simulink model "SSN_39busRT_Ctrl_4WT_19B"  (R2021a)
settings: Solver=ode3  StartTime=0.0  StopTime=10  FixedStep=Ts  MaxStep=1/60  RelTol=1e-2  AbsTol=1e-1
PreLoadFcn:
  | Ts=2.50e-6; ssn_ieee39_params; load('Pwf.mat');
InitFcn:
  | Ts=2.50e-6; ssn_ieee39_params; load('Pwf.mat');
values from neighbouring files (symbols this model uses):
  f = 50    [ssn_ieee39_params_ctrl.m]
  fNom = f    (= 60)    [ssn_ieee39_params_ctrl.m]
  ILR = 5.02    [ssn_ieee39_params_ctrl.m]
  IQMIN = 0.1    [ssn_ieee39_params_ctrl.m]
  ISCLIM = 1    [ssn_ieee39_params_ctrl.m]
  ITFpu = 1.10    (= 1.1)    [ssn_ieee39_params_ctrl.m]
  K = 1    [ssn_ieee39_params_ctrl.m]
  K1 = 1    [ssn_ieee39_params_ctrl.m]
  K2 = 2    [ssn_ieee39_params_ctrl.m]
  KCL = 1.04    [ssn_ieee39_params_ctrl.m]
  KFB = 0    [ssn_ieee39_params_ctrl.m]
  KFF = 1    [ssn_ieee39_params_ctrl.m]
  KFIX = 1    [ssn_ieee39_params_ctrl.m]
  KG = 1    [ssn_ieee39_params_ctrl.m]
  KIA = 59.91    [ssn_ieee39_params_ctrl.m]
  KIOEX = 0.0303    [ssn_ieee39_params_ctrl.m]
  KIUEX = 0.0303    [ssn_ieee39_params_ctrl.m]
  KIUOEX = 1    [ssn_ieee39_params_ctrl.m]
  KIUUEX = 1    [ssn_ieee39_params_ctrl.m]
  KLR = 22.47    [ssn_ieee39_params_ctrl.m]
  KM = 1    [ssn_ieee39_params_ctrl.m]
  KOEL = 0.24    [ssn_ieee39_params_ctrl.m]
  Kp = 1    [ssn_ieee39_params_ctrl.m]
  KPA = 30    [ssn_ieee39_params_ctrl.m]
  KPOEL = 1    [ssn_ieee39_params_ctrl.m]
  KPOEX = 0    [ssn_ieee39_params_ctrl.m]
  KPUEX = 0    [ssn_ieee39_params_ctrl.m]
  KSCALE = 0.319    [ssn_ieee39_params_ctrl.m]
  KUF = 0    [ssn_ieee39_params_ctrl.m]
  KUI = 0.001    [ssn_ieee39_params_ctrl.m]
  KUL = 0.24    [ssn_ieee39_params_ctrl.m]
  s = 10    [ssn_ieee39_params_ctrl.m]
  TA = 0.01    [ssn_ieee39_params_ctrl.m]
  Tadj = 0    [ssn_ieee39_params_ctrl.m]
  taps = [1 1 1.07 1.07 1.009 1.025 1 1.025 1.025 1.025]*1    [ssn_ieee39_params_ctrl.m]
  TF = 0.02    [ssn_ieee39_params_ctrl.m]
  TG = 0.024    [ssn_ieee39_params_ctrl.m]
  TINV = 0    [ssn_ieee39_params_ctrl.m]
  TIT = 0.1    [ssn_ieee39_params_ctrl.m]
  TL_10_11_len = 14    [ssn_ieee39_params_ctrl.m]
  TL_10_13_len = 14    [ssn_ieee39_params_ctrl.m]
  TL_13_14_len = 32    [ssn_ieee39_params_ctrl.m]
  TL_14_15_len = 70    [ssn_ieee39_params_ctrl.m]
  TL_15_16_len = 31.5    [ssn_ieee39_params_ctrl.m]
  TL_16_17_len = 26    [ssn_ieee39_params_ctrl.m]
  TL_16_19_len = 61    [ssn_ieee39_params_ctrl.m]
  TL_16_21_len = 46    [ssn_ieee39_params_ctrl.m]
  TL_16_24_len = 15    [ssn_ieee39_params_ctrl.m]
  TL_17_18_len = 26    [ssn_ieee39_params_ctrl.m]
  TL_17_27_len = 59    [ssn_ieee39_params_ctrl.m]
  TL_1_2_len = 134    [ssn_ieee39_params_ctrl.m]
  TL_1_39_len = 105    [ssn_ieee39_params_ctrl.m]
  TL_21_22_len = 47    [ssn_ieee39_params_ctrl.m]
  TL_22_23_len = 33    [ssn_ieee39_params_ctrl.m]
  TL_24_23_len = 88    [ssn_ieee39_params_ctrl.m]
  TL_25_26_len = 101    [ssn_ieee39_params_ctrl.m]
  TL_26_27_len = 46.5    [ssn_ieee39_params_ctrl.m]
  TL_26_28_len = 151    [ssn_ieee39_params_ctrl.m]
  TL_26_29_len = 200    [ssn_ieee39_params_ctrl.m]
  TL_28_29_len = 48    [ssn_ieee39_params_ctrl.m]
  TL_2_25_len = 28    [ssn_ieee39_params_ctrl.m]
  TL_2_2_len = 49    [ssn_ieee39_params_ctrl.m]
  TL_3_18_len = 42    [ssn_ieee39_params_ctrl.m]
  TL_3_4_len = 53    [ssn_ieee39_params_ctrl.m]
  TL_4_14_len = 33    [ssn_ieee39_params_ctrl.m]
  TL_4_5_len = 32.5    [ssn_ieee39_params_ctrl.m]
  TL_5_6_len = 14    [ssn_ieee39_params_ctrl.m]
  TL_5_8_len = 32    [ssn_ieee39_params_ctrl.m]
  TL_6_11_len = 26.5    [ssn_ieee39_params_ctrl.m]
  TL_6_7_len = 25.5    [ssn_ieee39_params_ctrl.m]
  TL_7_8_len = 15    [ssn_ieee39_params_ctrl.m]
  TL_8_9_len = 93    [ssn_ieee39_params_ctrl.m]
  TL_9_39_len = 136    [ssn_ieee39_params_ctrl.m]
  TOEL = 5.00    (= 5)    [ssn_ieee39_params_ctrl.m]
  TQREF = 0    [ssn_ieee39_params_ctrl.m]
  TQSCL = 0.012    [ssn_ieee39_params_ctrl.m]
  Ts_PMU = 1/1000    (= 0.001)    [ssn_ieee39_params_ctrl.m]
  TU1 = 0    [ssn_ieee39_params_ctrl.m]
  TU2 = 0    [ssn_ieee39_params_ctrl.m]
  TU3 = 0    [ssn_ieee39_params_ctrl.m]
  TU4 = 0    [ssn_ieee39_params_ctrl.m]
  TUL = 0    [ssn_ieee39_params_ctrl.m]
  TUP = 0.050    (= 0.05)    [ssn_ieee39_params_ctrl.m]
  TUQ = .005    (= 0.005)    [ssn_ieee39_params_ctrl.m]
  TUV = 0.2    [ssn_ieee39_params_ctrl.m]
  VAAMAX = VAMAX    (= 7.05)    [ssn_ieee39_params_ctrl.m]
  VAMAX = 7.05    [ssn_ieee39_params_ctrl.m]
  VAMIN = -6.11    [ssn_ieee39_params_ctrl.m]
  VBMAX = 999    [ssn_ieee39_params_ctrl.m]
  VF = 0    [ssn_ieee39_params_ctrl.m]
  VFB = 0    [ssn_ieee39_params_ctrl.m]
  VMMAX = 7.05    [ssn_ieee39_params_ctrl.m]
  VMMIN = -6.11    [ssn_ieee39_params_ctrl.m]
  VOELmax1 = 0.2353    [ssn_ieee39_params_ctrl.m]
  VOELmax2 = 0.0    (= 0)    [ssn_ieee39_params_ctrl.m]
  VOELmin1 = -0.24    [ssn_ieee39_params_ctrl.m]
  VOELmin2 = -1.0    (= -1)    [ssn_ieee39_params_ctrl.m]
  VRMAX = 7.05    [ssn_ieee39_params_ctrl.m]
  VRMIN = -6.11    [ssn_ieee39_params_ctrl.m]
  VSCLmax = 0.20    (= 0.2)    [ssn_ieee39_params_ctrl.m]
  VSCLmin = -0.10    (= -0.1)    [ssn_ieee39_params_ctrl.m]
  VUELmax1 = 1    [ssn_ieee39_params_ctrl.m]
  VUELmax2 = 1    [ssn_ieee39_params_ctrl.m]
  VUELmin1 = -1    [ssn_ieee39_params_ctrl.m]
  VUELmin2 = -1    [ssn_ieee39_params_ctrl.m]
  VUImax = 1    [ssn_ieee39_params_ctrl.m]
  VUImin = -1    [ssn_ieee39_params_ctrl.m]
undefined symbols (not defined in the file or in its folder): another_event_name, D1, Delta, DiscIntNeverNeededParam, find_system, MOV_segment9, my_event_name, powergui, Pw1, Pw2, Pw3, Pw4, vNomHV
libraries: powerlib_extras x162, spsThreePhaseVIMeasurementLib x55, spsCurrentMeasurementLib x52, simulink_extras x44, slpidlib x40, op_dpl_lib x36, spsST2AModel x20, spsThreePhaseParallelRLCLoadLib x20, spsThreePhaseTransformerTwoWindingsLib x17, spsControlledVoltageSourceLib x16, spsVoltageMeasurementLib x12, spsSynchronousMachinepuStandardLib x10
(part 2 of 19)

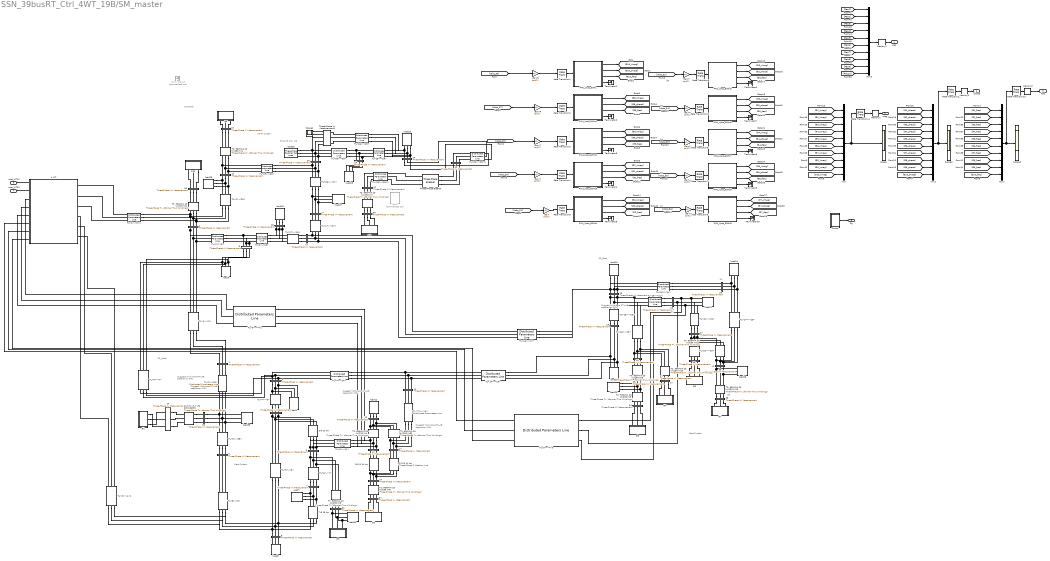
== system SSN_39busRT_Ctrl_4WT_19B/SM_master ==
  note: SS_East
  note: SM_North
  note: SS_West
  note: West System
  note: Suggest multi-core
      | RT-LAB separation DPL
  note: Suggest Multi-core
      | RT-LAB separation DPL
  note: Suggest Multi-core
      | RT-LAB separation DPL
  note: Suggest Multi-core
      | RT-LAB separation DPL
  note: P&Q 29 ==> 26
  note: North System
  note: 33
  note: 21
  note: 24
  note: 36
  note: 23
  note: Suggest Multi-core
      | RT-LAB separation DPL
  note: East System
  note: G3
  note: G7
  note: G6
  note: G4
  note: G5
  1 : spsThreePhaseVIMeasurementLib/Three-Phase V-I Measurement  VoltageMeasurement=phase-to-phase  SetLabelV=on  LabelV=Vabc_1  Vpu=off  VpuLL=on  CurrentMeasurement=no  SetLabelI=on  LabelI=Iabc_B2  Ipu=off  Pbase=100e6  Vbase=Bus(1,2)*1e3  OutputType=Complex  PhasorSimulation=off  PSBequivalent=0
  10 : spsThreePhaseVIMeasurementLib/Three-Phase V-I Measurement  VoltageMeasurement=phase-to-phase  SetLabelV=on  LabelV=Vabc_10  Vpu=off  VpuLL=on  CurrentMeasurement=no  SetLabelI=on  LabelI=Iabc_B2  Ipu=off  Pbase=100e6  Vbase=Bus(10,2)*1e3  OutputType=Complex  PhasorSimulation=off  PSBequivalent=0
  10-11 14 km : spsThreePhasePISectionLineLib/Three-Phase PI Section Line  LConnTagsString=a|b|c  RConnTagsString=A|B|C  Length=TL_10_11_len  Frequency=60  Resistances=[0.476 1.904]/TL_10_11_len  Inductances="[0.014  0.04]/TL_10_11_len"  Capacitances=[0.162e-6 0.074e-6]/TL_10_11_len
  10-13 14 km : spsThreePhasePISectionLineLib/Three-Phase PI Section Line  LConnTagsString=a|b|c  RConnTagsString=A|B|C  Length=TL_10_13_len  Frequency=60  Resistances=[0.476 1.904]/TL_10_13_len  Inductances="[0.014  0.04]/TL_10_13_len"  Capacitances=[0.162e-6 0.074e-6]/TL_10_13_len
  11 : spsThreePhaseVIMeasurementLib/Three-Phase V-I Measurement  VoltageMeasurement=phase-to-phase  SetLabelV=on  LabelV=Vabc_11  Vpu=off  VpuLL=on  CurrentMeasurement=no  SetLabelI=on  LabelI=Iabc_B2  Ipu=off  Pbase=100e6  Vbase=Bus(11,2)*1e3  OutputType=Complex  PhasorSimulation=off  PSBequivalent=0
  12 : spsThreePhaseVIMeasurementLib/Three-Phase V-I Measurement  VoltageMeasurement=phase-to-phase  SetLabelV=on  LabelV=Vabc_12  Vpu=off  VpuLL=on  CurrentMeasurement=no  SetLabelI=on  LabelI=Iabc_B2  Ipu=off  Pbase=100e6  Vbase=Bus(12,2)*1e3  OutputType=Complex  PhasorSimulation=off  PSBequivalent=0
  13 : spsThreePhaseVIMeasurementLib/Three-Phase V-I Measurement  VoltageMeasurement=phase-to-phase  SetLabelV=on  LabelV=Vabc_13  Vpu=off  VpuLL=on  CurrentMeasurement=no  SetLabelI=on  LabelI=Iabc_B2  Ipu=off  Pbase=100e6  Vbase=Bus(13,2)*1e3  OutputType=Complex  PhasorSimulation=off  PSBequivalent=0
  14 : spsThreePhaseVIMeasurementLib/Three-Phase V-I Measurement  VoltageMeasurement=phase-to-phase  SetLabelV=on  LabelV=Vabc_14  Vpu=off  VpuLL=on  CurrentMeasurement=no  SetLabelI=on  LabelI=Iabc_B2  Ipu=off  Pbase=100e6  Vbase=Bus(14,2)*1e3  OutputType=Complex  PhasorSimulation=off  PSBequivalent=0
  15 : spsThreePhaseVIMeasurementLib/Three-Phase V-I Measurement  VoltageMeasurement=phase-to-phase  SetLabelV=on  LabelV=Vabc_15  Vpu=off  VpuLL=on  CurrentMeasurement=no  SetLabelI=on  LabelI=Iabc_B2  Ipu=off  Pbase=100e6  Vbase=Bus(15,2)*1e3  OutputType=Complex  PhasorSimulation=off  PSBequivalent=0
  16 : spsThreePhaseVIMeasurementLib/Three-Phase V-I Measurement  VoltageMeasurement=phase-to-phase  SetLabelV=on  LabelV=Vabc_16  Vpu=off  VpuLL=on  CurrentMeasurement=no  SetLabelI=on  LabelI=Iabc_B2  Ipu=off  Pbase=100e6  Vbase=Bus(16,2)*1e3  OutputType=Complex  PhasorSimulation=off  PSBequivalent=0
  17 : spsThreePhaseVIMeasurementLib/Three-Phase V-I Measurement  VoltageMeasurement=phase-to-phase  SetLabelV=on  LabelV=Vabc_17  Vpu=off  VpuLL=on  CurrentMeasurement=no  SetLabelI=on  LabelI=Iabc_B2  Ipu=off  Pbase=100e6  Vbase=Bus(17,2)*1e3  OutputType=Complex  PhasorSimulation=off  PSBequivalent=0
  18 : spsThreePhaseVIMeasurementLib/Three-Phase V-I Measurement  VoltageMeasurement=phase-to-phase  SetLabelV=on  LabelV=Vabc_18  Vpu=off  VpuLL=on  CurrentMeasurement=no  SetLabelI=on  LabelI=Iabc_B2  Ipu=off  Pbase=100e6  Vbase=Bus(18,2)*1e3  OutputType=Complex  PhasorSimulation=off  PSBequivalent=0
  19 : spsThreePhaseVIMeasurementLib/Three-Phase V-I Measurement  VoltageMeasurement=phase-to-phase  SetLabelV=on  LabelV=Vabc_19  Vpu=off  VpuLL=on  CurrentMeasurement=no  SetLabelI=on  LabelI=Iabc_B2  Ipu=off  Pbase=100e6  Vbase=Bus(19,2)*1e3  OutputType=Complex  PhasorSimulation=off  PSBequivalent=0
  2 : spsThreePhaseVIMeasurementLib/Three-Phase V-I Measurement  VoltageMeasurement=phase-to-phase  SetLabelV=on  LabelV=Vabc_2  Vpu=off  VpuLL=on  CurrentMeasurement=no  SetLabelI=on  LabelI=Iabc_B2  Ipu=off  Pbase=100e6  Vbase=Bus(2,2)*1e3  OutputType=Complex  PhasorSimulation=off  PSBequivalent=0
  20 : spsThreePhaseVIMeasurementLib/Three-Phase V-I Measurement  VoltageMeasurement=phase-to-phase  SetLabelV=on  LabelV=Vabc_20  Vpu=off  VpuLL=on  CurrentMeasurement=no  SetLabelI=on  LabelI=Iabc_B2  Ipu=off  Pbase=100e6  Vbase=Bus(20,2)*1e3  OutputType=Complex  PhasorSimulation=off  PSBequivalent=0
  21 : spsThreePhaseVIMeasurementLib/Three-Phase V-I Measurement  VoltageMeasurement=phase-to-phase  SetLabelV=on  LabelV=Vabc_33  Vpu=off  VpuLL=on  CurrentMeasurement=yes  SetLabelI=on  LabelI=Iabc_33  Ipu=on  Pbase=1000e6  Vbase=Bus(33,2)*1e3  OutputType=Complex  PhasorSimulation=off  PSBequivalent=0
  22 : spsThreePhaseVIMeasurementLib/Three-Phase V-I Measurement  VoltageMeasurement=phase-to-phase  SetLabelV=on  LabelV=Vabc_22  Vpu=off  VpuLL=on  CurrentMeasurement=no  SetLabelI=on  LabelI=Iabc_B2  Ipu=off  Pbase=100e6  Vbase=Bus(22,2)*1e3  OutputType=Complex  PhasorSimulation=off  PSBequivalent=0
  23 : spsThreePhaseVIMeasurementLib/Three-Phase V-I Measurement  VoltageMeasurement=phase-to-phase  SetLabelV=on  LabelV=Vabc_21  Vpu=off  VpuLL=on  CurrentMeasurement=no  SetLabelI=on  LabelI=Iabc_B2  Ipu=off  Pbase=100e6  Vbase=Bus(21,2)*1e3  OutputType=Complex  PhasorSimulation=off  PSBequivalent=0
  24 : spsThreePhaseVIMeasurementLib/Three-Phase V-I Measurement  VoltageMeasurement=phase-to-phase  SetLabelV=on  LabelV=Vabc_391  Vpu=off  VpuLL=on  CurrentMeasurement=yes  SetLabelI=on  LabelI=Iabc_391  Ipu=on  Pbase=1000e6  Vbase=Bus(30,2)*1e3  OutputType=Complex  PhasorSimulation=off  PSBequivalent=0
  25 : spsThreePhaseVIMeasurementLib/Three-Phase V-I Measurement  VoltageMeasurement=phase-to-phase  SetLabelV=on  LabelV=Vabc_25  Vpu=off  VpuLL=on  CurrentMeasurement=no  SetLabelI=on  LabelI=Iabc_B2  Ipu=off  Pbase=100e6  Vbase=Bus(25,2)*1e3  OutputType=Complex  PhasorSimulation=off  PSBequivalent=0
  26 : spsThreePhaseVIMeasurementLib/Three-Phase V-I Measurement  VoltageMeasurement=phase-to-phase  SetLabelV=on  LabelV=Vabc_26  Vpu=off  VpuLL=on  CurrentMeasurement=no  SetLabelI=on  LabelI=Iabc_B2  Ipu=off  Pbase=100e6  Vbase=Bus(26,2)*1e3  OutputType=Complex  PhasorSimulation=off  PSBequivalent=0
  27 : spsThreePhaseVIMeasurementLib/Three-Phase V-I Measurement  VoltageMeasurement=phase-to-phase  SetLabelV=on  LabelV=Vabc_27  Vpu=off  VpuLL=on  CurrentMeasurement=no  SetLabelI=on  LabelI=Iabc_B2  Ipu=off  Pbase=100e6  Vbase=Bus(27,2)*1e3  OutputType=Complex  PhasorSimulation=off  PSBequivalent=0
  28 : spsThreePhaseVIMeasurementLib/Three-Phase V-I Measurement  VoltageMeasurement=phase-to-phase  SetLabelV=on  LabelV=Vabc_28  Vpu=off  VpuLL=on  CurrentMeasurement=no  SetLabelI=on  LabelI=Iabc_B2  Ipu=off  Pbase=100e6  Vbase=Bus(28,2)*1e3  OutputType=Complex  PhasorSimulation=off  PSBequivalent=0
  29 : spsThreePhaseVIMeasurementLib/Three-Phase V-I Measurement  VoltageMeasurement=phase-to-phase  SetLabelV=on  LabelV=Vabc_29  Vpu=off  VpuLL=on  CurrentMeasurement=no  SetLabelI=on  LabelI=Iabc_B2  Ipu=off  Pbase=100e6  Vbase=Bus(29,2)*1e3  OutputType=Complex  PhasorSimulation=off  PSBequivalent=0
  3 : spsThreePhaseVIMeasurementLib/Three-Phase V-I Measurement  VoltageMeasurement=phase-to-phase  SetLabelV=on  LabelV=Vabc_B3  Vpu=off  VpuLL=on  CurrentMeasurement=yes  SetLabelI=on  LabelI=Iabc_B3  Ipu=off  Pbase=100e6  Vbase=Bus(3,2)*1e3  OutputType=Complex  PhasorSimulation=off  PSBequivalent=0
  30 : spsThreePhaseVIMeasurementLib/Three-Phase V-I Measurement  VoltageMeasurement=phase-to-phase  SetLabelV=on  LabelV=Vabc_30  Vpu=off  VpuLL=on  CurrentMeasurement=yes  SetLabelI=on  LabelI=Iabc_30  Ipu=on  Pbase=1000e6  Vbase=Bus(30,2)*1e3  OutputType=Complex  PhasorSimulation=off  PSBequivalent=0
  31 : spsThreePhaseVIMeasurementLib/Three-Phase V-I Measurement  VoltageMeasurement=phase-to-phase  SetLabelV=on  LabelV=Vabc_31  Vpu=off  VpuLL=on  CurrentMeasurement=yes  SetLabelI=on  LabelI=Iabc_31  Ipu=on  Pbase=1000e6  Vbase=Bus(31,2)*1e3  OutputType=Complex  PhasorSimulation=off  PSBequivalent=0
  32 : spsThreePhaseVIMeasurementLib/Three-Phase V-I Measurement  VoltageMeasurement=phase-to-phase  SetLabelV=on  LabelV=Vabc_32  Vpu=off  VpuLL=on  CurrentMeasurement=yes  SetLabelI=on  LabelI=Iabc_32  Ipu=on  Pbase=1000e6  Vbase=Bus(32,2)*1e3  OutputType=Complex  PhasorSimulation=off  PSBequivalent=0
  33 : spsThreePhaseVIMeasurementLib/Three-Phase V-I Measurement  VoltageMeasurement=phase-to-phase  SetLabelV=on  LabelV=Vabc_24  Vpu=off  VpuLL=on  CurrentMeasurement=no  SetLabelI=on  LabelI=Iabc_B2  Ipu=off  Pbase=100e6  Vbase=Bus(24,2)*1e3  OutputType=Complex  PhasorSimulation=off  PSBequivalent=0
  34 : spsThreePhaseVIMeasurementLib/Three-Phase V-I Measurement  VoltageMeasurement=phase-to-phase  SetLabelV=on  LabelV=Vabc_34  Vpu=off  VpuLL=on  CurrentMeasurement=yes  SetLabelI=on  LabelI=Iabc_34  Ipu=on  Pbase=1000e6  Vbase=Bus(34,2)*1e3  OutputType=Complex  PhasorSimulation=off  PSBequivalent=0
  35 : spsThreePhaseVIMeasurementLib/Three-Phase V-I Measurement  VoltageMeasurement=phase-to-phase  SetLabelV=on  LabelV=Vabc_36  Vpu=off  VpuLL=on  CurrentMeasurement=yes  SetLabelI=on  LabelI=Iabc_36  Ipu=on  Pbase=1000e6  Vbase=Bus(36,2)*1e3  OutputType=Complex  PhasorSimulation=off  PSBequivalent=0
  35. : spsThreePhaseVIMeasurementLib/Three-Phase V-I Measurement  VoltageMeasurement=phase-to-phase  SetLabelV=on  LabelV=Vabc_35  Vpu=off  VpuLL=on  CurrentMeasurement=yes  SetLabelI=on  LabelI=Iabc_35  Ipu=on  Pbase=1000e6  Vbase=Bus(35,2)*1e3  OutputType=Complex  PhasorSimulation=off  PSBequivalent=0
  36 : spsThreePhaseVIMeasurementLib/Three-Phase V-I Measurement  VoltageMeasurement=phase-to-phase  SetLabelV=on  LabelV=Vabc_23  Vpu=off  VpuLL=on  CurrentMeasurement=no  SetLabelI=on  LabelI=Iabc_B2  Ipu=off  Pbase=100e6  Vbase=Bus(23,2)*1e3  OutputType=Complex  PhasorSimulation=off  PSBequivalent=0
  37 : spsThreePhaseVIMeasurementLib/Three-Phase V-I Measurement  VoltageMeasurement=phase-to-phase  SetLabelV=on  LabelV=Vabc_37  Vpu=off  VpuLL=on  CurrentMeasurement=yes  SetLabelI=on  LabelI=Iabc_37  Ipu=on  Pbase=1000e6  Vbase=Bus(37,2)*1e3  OutputType=Complex  PhasorSimulation=off  PSBequivalent=0
  38 : spsThreePhaseVIMeasurementLib/Three-Phase V-I Measurement  VoltageMeasurement=phase-to-phase  SetLabelV=on  LabelV=Vabc_38  Vpu=off  VpuLL=on  CurrentMeasurement=yes  SetLabelI=on  LabelI=Iabc_38  Ipu=on  Pbase=1000e6  Vbase=Bus(38,2)*1e3  OutputType=Complex  PhasorSimulation=off  PSBequivalent=0
  39 : spsThreePhaseVIMeasurementLib/Three-Phase V-I Measurement  VoltageMeasurement=phase-to-phase  SetLabelV=on  LabelV=Vabc_39  Vpu=off  VpuLL=on  CurrentMeasurement=no  SetLabelI=on  LabelI=Iabc_B2  Ipu=off  Pbase=100e6  Vbase=Bus(39,2)*1e3  OutputType=Complex  PhasorSimulation=off  PSBequivalent=0
  4 : spsThreePhaseVIMeasurementLib/Three-Phase V-I Measurement  VoltageMeasurement=phase-to-phase  SetLabelV=on  LabelV=Vabc_B4  Vpu=off  VpuLL=on  CurrentMeasurement=yes  SetLabelI=on  LabelI=Iabc_B4  Ipu=off  Pbase=100e6  Vbase=Bus(4,2)*1e3  OutputType=Complex  PhasorSimulation=off  PSBequivalent=0
  4 WT : Subsystem
  40 : spsThreePhaseVIMeasurementLib/Three-Phase V-I Measurement  VoltageMeasurement=phase-to-phase  SetLabelV=on  LabelV=Vabc_40  Vpu=off  VpuLL=on  CurrentMeasurement=no  SetLabelI=on  LabelI=Iabc_B2  Ipu=off  Pbase=100e6  Vbase=Bus(29,2)*1e3  OutputType=Complex  PhasorSimulation=off  PSBequivalent=0
  41 : spsThreePhaseVIMeasurementLib/Three-Phase V-I Measurement  VoltageMeasurement=phase-to-phase  SetLabelV=on  LabelV=Vabc_41  Vpu=off  VpuLL=on  CurrentMeasurement=no  SetLabelI=on  LabelI=Iabc_B2  Ipu=off  Pbase=100e6  Vbase=Bus(25,2)*1e3  OutputType=Complex  PhasorSimulation=off  PSBequivalent=0
  5 : spsThreePhaseVIMeasurementLib/Three-Phase V-I Measurement  VoltageMeasurement=phase-to-phase  SetLabelV=on  LabelV=Vabc_5  Vpu=off  VpuLL=on  CurrentMeasurement=no  SetLabelI=on  LabelI=Iabc_B2  Ipu=off  Pbase=100e6  Vbase=Bus(5,2)*1e3  OutputType=Complex  PhasorSimulation=off  PSBequivalent=0
  5-6 14 km : spsThreePhasePISectionLineLib/Three-Phase PI Section Line  LConnTagsString=a|b|c  RConnTagsString=A|B|C  Length=TL_5_6_len  Frequency=60  Resistances=[0.476 1.904]/TL_5_6_len  Inductances=[0.014 0.04]/TL_5_6_len  Capacitances=[0.162e-6 0.074e-6]/TL_5_6_len
  6 : spsThreePhaseVIMeasurementLib/Three-Phase V-I Measurement  VoltageMeasurement=phase-to-phase  SetLabelV=on  LabelV=Vabc_6  Vpu=off  VpuLL=on  CurrentMeasurement=no  SetLabelI=on  LabelI=Iabc_B2  Ipu=off  Pbase=100e6  Vbase=Bus(6,2)*1e3  OutputType=Complex  PhasorSimulation=off  PSBequivalent=0
  7 : spsThreePhaseVIMeasurementLib/Three-Phase V-I Measurement  VoltageMeasurement=phase-to-phase  SetLabelV=on  LabelV=Vabc_7  Vpu=off  VpuLL=on  CurrentMeasurement=no  SetLabelI=on  LabelI=Iabc_B2  Ipu=off  Pbase=100e6  Vbase=Bus(8,2)*1e3  OutputType=Complex  PhasorSimulation=off  PSBequivalent=0
  7-8 15 km : spsThreePhasePISectionLineLib/Three-Phase PI Section Line  LConnTagsString=a|b|c  RConnTagsString=A|B|C  Length=TL_7_8_len  Frequency=60  Resistances=[0.476 1.904]/TL_7_8_len  Inductances="[0.015  0.044]/TL_7_8_len"  Capacitances=[0.174e-6 0.079e-6]/TL_7_8_len
  8 : spsThreePhaseVIMeasurementLib/Three-Phase V-I Measurement  VoltageMeasurement=phase-to-phase  SetLabelV=on  LabelV=Vabc_8  Vpu=off  VpuLL=on  CurrentMeasurement=no  SetLabelI=on  LabelI=Iabc_B2  Ipu=off  Pbase=100e6  Vbase=Bus(8,2)*1e3  OutputType=Complex  PhasorSimulation=off  PSBequivalent=0
  9 : spsThreePhaseVIMeasurementLib/Three-Phase V-I Measurement  VoltageMeasurement=phase-to-phase  SetLabelV=on  LabelV=Vabc_9  Vpu=off  VpuLL=on  CurrentMeasurement=no  SetLabelI=on  LabelI=Iabc_B2  Ipu=off  Pbase=100e6  Vbase=Bus(9,2)*1e3  OutputType=Complex  PhasorSimulation=off  PSBequivalent=0
  G1 : Subsystem
  G10 : Subsystem
  G2 : Subsystem
  G3 : Subsystem
  G4 : Subsystem
  G5 : Subsystem
  G6 : Subsystem
  G7 : Subsystem
  G8 : Subsystem
  G9 : Subsystem
  Gain{,1..9} (10 alike) : Gain  Gain=sqrt(2)
  Memory{1..4} (4 alike) : Memory
  Mux{,1..3} (4 alike) : Mux  Inputs=10
  PMU_Vpos_60Hz : Subsystem  AncestorBlock=|  DialogController=POWERSYS.PowerSysDialog  mask(Discrete 3-phase Positive-sequence fundamental value){Freq=60, Par_Init=[0 angle(10)], Ts=Ts_PMU}
      | powerlib_extras/Discrete
      | Measurements/Discrete 3-phase
      | Positive-Sequence
      | Fundamental Value
      mask prompts: Freq "Fundamental frequency (Hz):"; Par_Init "Initial input (positive component): [ Mag  Phase(degrees) ]"; Ts "Sample time:"
      mask help:
      | Compute the positive-sequence component of the input signal at the given fundamental frequency. The input is set of three balanced or unbalanced signals which may contain harmonics.
      |
      | The two outputs return respectively the magnitude (same units as the input signal) and phase (in degrees) of the fundamental.
      |
      | For the first cycle of simulation, the outputs are held constant to the values specified by the Initial input parameter.
      mask init:
      | SamplesPerCycle=1/Freq/Ts;
      | RoundSamplesPerCycle=round(SamplesPerCycle);
      | Delay=RoundSamplesPerCycle*Ts - Ts/2;
      | Correction=SamplesPerCycle/RoundSamplesPerCycle - 1;
      | Real_Init=Par_Init(1)*cos(pi/180*Par_Init(2));
      | Imag_Init=Par_Init(1)*sin(pi/180*Par_Init(2));
      | power_initmask();
      mask Help: This block is part of a subset of blocks in the Extras library that does not have documentation associated with it, other than the block mask description.
      mask Display: disp('')
  PMU_Vpos_60Hz1 : Subsystem  AncestorBlock=|  DialogController=POWERSYS.PowerSysDialog  mask(Discrete 3-phase Positive-sequence fundamental value){Freq=60, Par_Init=[0 angle(8)], Ts=Ts_PMU}
      | powerlib_extras/Discrete
      | Measurements/Discrete 3-phase
      | Positive-Sequence
      | Fundamental Value
      mask prompts: Freq "Fundamental frequency (Hz):"; Par_Init "Initial input (positive component): [ Mag  Phase(degrees) ]"; Ts "Sample time:"
      mask help:
      | Compute the positive-sequence component of the input signal at the given fundamental frequency. The input is set of three balanced or unbalanced signals which may contain harmonics.
      |
      | The two outputs return respectively the magnitude (same units as the input signal) and phase (in degrees) of the fundamental.
      |
      | For the first cycle of simulation, the outputs are held constant to the values specified by the Initial input parameter.
      mask init: same as SSN_39busRT_Ctrl_4WT_19B/SM_master/PMU_Vpos_60Hz
      mask Help: This block is part of a subset of blocks in the Extras library that does not have documentation associated with it, other than the block mask description.
      mask Display: disp('')
  PMU_Vpos_60Hz2 : Subsystem  AncestorBlock=|  DialogController=POWERSYS.PowerSysDialog  mask(Discrete 3-phase Positive-sequence fundamental value){Freq=60, Par_Init=[0 angle(9)], Ts=Ts_PMU}
      | powerlib_extras/Discrete
      | Measurements/Discrete 3-phase
      | Positive-Sequence
      | Fundamental Value
      mask prompts: Freq "Fundamental frequency (Hz):"; Par_Init "Initial input (positive component): [ Mag  Phase(degrees) ]"; Ts "Sample time:"
      mask help:
      | Compute the positive-sequence component of the input signal at the given fundamental frequency. The input is set of three balanced or unbalanced signals which may contain harmonics.
      |
      | The two outputs return respectively the magnitude (same units as the input signal) and phase (in degrees) of the fundamental.
      |
      | For the first cycle of simulation, the outputs are held constant to the values specified by the Initial input parameter.
      mask init: same as SSN_39busRT_Ctrl_4WT_19B/SM_master/PMU_Vpos_60Hz
      mask Help: This block is part of a subset of blocks in the Extras library that does not have documentation associated with it, other than the block mask description.
      mask Display: disp('')
  PMU_Vpos_60Hz3 : Subsystem  AncestorBlock=|  DialogController=POWERSYS.PowerSysDialog  mask(Discrete 3-phase Positive-sequence fundamental value){Freq=60, Par_Init=[0 angle(1)], Ts=Ts_PMU}
      | powerlib_extras/Discrete
      | Measurements/Discrete 3-phase
      | Positive-Sequence
      | Fundamental Value
      mask prompts: Freq "Fundamental frequency (Hz):"; Par_Init "Initial input (positive component): [ Mag  Phase(degrees) ]"; Ts "Sample time:"
      mask help:
      | Compute the positive-sequence component of the input signal at the given fundamental frequency. The input is set of three balanced or unbalanced signals which may contain harmonics.
      |
      | The two outputs return respectively the magnitude (same units as the input signal) and phase (in degrees) of the fundamental.
      |
      | For the first cycle of simulation, the outputs are held constant to the values specified by the Initial input parameter.
      mask init: same as SSN_39busRT_Ctrl_4WT_19B/SM_master/PMU_Vpos_60Hz
      mask Help: This block is part of a subset of blocks in the Extras library that does not have documentation associated with it, other than the block mask description.
      mask Display: disp('')
  PMU_Vpos_60Hz4 : Subsystem  AncestorBlock=|  DialogController=POWERSYS.PowerSysDialog  mask(Discrete 3-phase Positive-sequence fundamental value){Freq=60, Par_Init=[0 angle(2)], Ts=Ts_PMU}
      | powerlib_extras/Discrete
      | Measurements/Discrete 3-phase
      | Positive-Sequence
      | Fundamental Value
      mask prompts: Freq "Fundamental frequency (Hz):"; Par_Init "Initial input (positive component): [ Mag  Phase(degrees) ]"; Ts "Sample time:"
      mask help:
      | Compute the positive-sequence component of the input signal at the given fundamental frequency. The input is set of three balanced or unbalanced signals which may contain harmonics.
      |
      | The two outputs return respectively the magnitude (same units as the input signal) and phase (in degrees) of the fundamental.
      |
      | For the first cycle of simulation, the outputs are held constant to the values specified by the Initial input parameter.
      mask init: same as SSN_39busRT_Ctrl_4WT_19B/SM_master/PMU_Vpos_60Hz
      mask Help: This block is part of a subset of blocks in the Extras library that does not have documentation associated with it, other than the block mask description.
      mask Display: disp('')
  PMU_Vpos_60Hz5 : Subsystem  AncestorBlock=|  DialogController=POWERSYS.PowerSysDialog  mask(Discrete 3-phase Positive-sequence fundamental value){Freq=fNom, Par_Init=[0 angle(3)], Ts=Ts_PMU}
      | powerlib_extras/Discrete
      | Measurements/Discrete 3-phase
      | Positive-Sequence
      | Fundamental Value
      mask prompts: Freq "Fundamental frequency (Hz):"; Par_Init "Initial input (positive component): [ Mag  Phase(degrees) ]"; Ts "Sample time:"
      mask help:
      | Compute the positive-sequence component of the input signal at the given fundamental frequency. The input is set of three balanced or unbalanced signals which may contain harmonics.
      |
      | The two outputs return respectively the magnitude (same units as the input signal) and phase (in degrees) of the fundamental.
      |
      | For the first cycle of simulation, the outputs are held constant to the values specified by the Initial input parameter.
      mask init: same as SSN_39busRT_Ctrl_4WT_19B/SM_master/PMU_Vpos_60Hz
      mask Help: This block is part of a subset of blocks in the Extras library that does not have documentation associated with it, other than the block mask description.
      mask Display: disp('')
  PMU_Vpos_60Hz6 : Subsystem  AncestorBlock=|  DialogController=POWERSYS.PowerSysDialog  mask(Discrete 3-phase Positive-sequence fundamental value){Freq=60, Par_Init=[0 angle(5)], Ts=Ts_PMU}
      | powerlib_extras/Discrete
      | Measurements/Discrete 3-phase
      | Positive-Sequence
      | Fundamental Value
      mask prompts: Freq "Fundamental frequency (Hz):"; Par_Init "Initial input (positive component): [ Mag  Phase(degrees) ]"; Ts "Sample time:"
      mask help:
      | Compute the positive-sequence component of the input signal at the given fundamental frequency. The input is set of three balanced or unbalanced signals which may contain harmonics.
      |
      | The two outputs return respectively the magnitude (same units as the input signal) and phase (in degrees) of the fundamental.
      |
      | For the first cycle of simulation, the outputs are held constant to the values specified by the Initial input parameter.
      mask init: same as SSN_39busRT_Ctrl_4WT_19B/SM_master/PMU_Vpos_60Hz
      mask Help: This block is part of a subset of blocks in the Extras library that does not have documentation associated with it, other than the block mask description.
      mask Display: disp('')
  PMU_Vpos_60Hz7 : Subsystem  AncestorBlock=|  DialogController=POWERSYS.PowerSysDialog  mask(Discrete 3-phase Positive-sequence fundamental value){Freq=60, Par_Init=[0 angle(4)], Ts=Ts_PMU}
      | powerlib_extras/Discrete
      | Measurements/Discrete 3-phase
      | Positive-Sequence
      | Fundamental Value
      mask prompts: Freq "Fundamental frequency (Hz):"; Par_Init "Initial input (positive component): [ Mag  Phase(degrees) ]"; Ts "Sample time:"
      mask help:
      | Compute the positive-sequence component of the input signal at the given fundamental frequency. The input is set of three balanced or unbalanced signals which may contain harmonics.
      |
      | The two outputs return respectively the magnitude (same units as the input signal) and phase (in degrees) of the fundamental.
      |
      | For the first cycle of simulation, the outputs are held constant to the values specified by the Initial input parameter.
      mask init: same as SSN_39busRT_Ctrl_4WT_19B/SM_master/PMU_Vpos_60Hz
      mask Help: This block is part of a subset of blocks in the Extras library that does not have documentation associated with it, other than the block mask description.
      mask Display: disp('')
  PMU_Vpos_60Hz8 : Subsystem  AncestorBlock=|  DialogController=POWERSYS.PowerSysDialog  mask(Discrete 3-phase Positive-sequence fundamental value){Freq=60, Par_Init=[0 angle(6)], Ts=Ts_PMU}
      | powerlib_extras/Discrete
      | Measurements/Discrete 3-phase
      | Positive-Sequence
      | Fundamental Value
      mask prompts: Freq "Fundamental frequency (Hz):"; Par_Init "Initial input (positive component): [ Mag  Phase(degrees) ]"; Ts "Sample time:"
      mask help:
      | Compute the positive-sequence component of the input signal at the given fundamental frequency. The input is set of three balanced or unbalanced signals which may contain harmonics.
      |
      | The two outputs return respectively the magnitude (same units as the input signal) and phase (in degrees) of the fundamental.
      |
      | For the first cycle of simulation, the outputs are held constant to the values specified by the Initial input parameter.
      mask init: same as SSN_39busRT_Ctrl_4WT_19B/SM_master/PMU_Vpos_60Hz
      mask Help: This block is part of a subset of blocks in the Extras library that does not have documentation associated with it, other than the block mask description.
      mask Display: disp('')
  PMU_Vpos_60Hz9 : Subsystem  AncestorBlock=|  DialogController=POWERSYS.PowerSysDialog  mask(Discrete 3-phase Positive-sequence fundamental value){Freq=60, Par_Init=[0 angle(7)], Ts=Ts_PMU}
      | powerlib_extras/Discrete
      | Measurements/Discrete 3-phase
      | Positive-Sequence
      | Fundamental Value
      mask prompts: Freq "Fundamental frequency (Hz):"; Par_Init "Initial input (positive component): [ Mag  Phase(degrees) ]"; Ts "Sample time:"
      mask help:
      | Compute the positive-sequence component of the input signal at the given fundamental frequency. The input is set of three balanced or unbalanced signals which may contain harmonics.
      |
      | The two outputs return respectively the magnitude (same units as the input signal) and phase (in degrees) of the fundamental.
      |
      | For the first cycle of simulation, the outputs are held constant to the values specified by the Initial input parameter.
      mask init: same as SSN_39busRT_Ctrl_4WT_19B/SM_master/PMU_Vpos_60Hz
      mask Help: This block is part of a subset of blocks in the Extras library that does not have documentation associated with it, other than the block mask description.
      mask Display: disp('')
  Power : Subsystem
  Rate Transition{1..10} (10 alike) : RateTransition  OutPortSampleTime=Ts_PMU
  Rate Transition11 : RateTransition  OutPortSampleTime=Ts
  Rate Transition12 : RateTransition  OutPortSampleTime=Ts
  Rate Transition13 : RateTransition  OutPortSampleTime=Ts
  Scope : Scope
  Scope1 : Scope  NumInputPorts=2
  Scope2 : Scope
  Scope3 : Scope
  T2: 900MVA 20 kV/230 kV1 : spsThreePhaseTransformerTwoWindingsLib/Three-Phase Transformer (Two Windings)  Winding1Connection=Delta (D1)  Winding2Connection=Yg  CoreType=Three single-phase transformers  SetSaturation=off  Hysteresis=off  DataFile='hysteresis'  SetInitialFlux=off  Measurements=None  UNITS=pu  NominalPower=[ 1000e6 60 ]  Winding1="[ 20e3*1.0 0.0003*s  0]"  Winding2="[ 345e3*taps(8) 0.0003*s  0.0232*s]"  Rm=500  Lm=500  L0=0.5  Saturation="[ 0,0  ;  0.005,1.2  ;  1.0,1.4 ]"  InitialFluxes=[ 0.8 , -0.8 , 0.7 ]  BreakLoop=off  DiscreteSolver=Trapezoidal iterative  DataType=off  TransfoNumber=0
  T2: 900MVA 20 kV/230 kV10 : spsThreePhaseTransformerTwoWindingsLib/Three-Phase Transformer (Two Windings)  Winding1Connection=Delta (D1)  Winding2Connection=Yg  CoreType=Three single-phase transformers  SetSaturation=off  Hysteresis=off  DataFile='hysteresis'  SetInitialFlux=off  Measurements=None  UNITS=pu  NominalPower=[ 1000e6 60 ]  Winding1="[ 20e3*1.0   0.00035*s  0]"  Winding2="[ 345e3*taps(4)  0.00035*s  0.0142*s]"  Rm=500  Lm=500  L0=0.5  Saturation="[ 0,0  ;  0.005,1.2  ;  1.0,1.4 ]"  InitialFluxes=[ 0.8 , -0.8 , 0.7 ]  BreakLoop=off  DiscreteSolver=Trapezoidal iterative  DataType=off  TransfoNumber=0
  T2: 900MVA 20 kV/230 kV11 : spsThreePhaseTransformerTwoWindingsLib/Three-Phase Transformer (Two Windings)  Winding1Connection=Delta (D1)  Winding2Connection=Yg  CoreType=Three single-phase transformers  SetSaturation=off  Hysteresis=off  DataFile='hysteresis'  SetInitialFlux=off  Measurements=None  UNITS=pu  NominalPower=[ 1000e6 60 ]  Winding1="[ 20e3*1.0  1e-6  0]"  Winding2="[ 345e3*taps(6)  1e-6  0.0143*s]"  Rm=500  Lm=500  L0=0.5  Saturation="[ 0,0  ;  0.005,1.2  ;  1.0,1.4 ]"  InitialFluxes=[ 0.8 , -0.8 , 0.7 ]  BreakLoop=off  DiscreteSolver=Trapezoidal iterative  DataType=off  TransfoNumber=0
  T2: 900MVA 20 kV/230 kV12 : spsThreePhaseTransformerTwoWindingsLib/Three-Phase Transformer (Two Windings)  Winding1Connection=Delta (D1)  Winding2Connection=Yg  CoreType=Three single-phase transformers  SetSaturation=off  Hysteresis=off  DataFile='hysteresis'  SetInitialFlux=off  Measurements=None  UNITS=pu  NominalPower=[ 1000e6 60 ]  Winding1="[ 20e3    0.00025*s  0.0]"  Winding2="[ 345e3*taps(7)    0.00025*s  0.0272*s]"  Rm=500  Lm=500  L0=0.5  Saturation="[ 0,0  ;  0.005,1.2  ;  1.0,1.4 ]"  InitialFluxes=[ 0.8 , -0.8 , 0.7 ]  BreakLoop=off  DiscreteSolver=Trapezoidal iterative  DataType=off  TransfoNumber=0
  T2: 900MVA 20 kV/230 kV2 : spsThreePhaseTransformerTwoWindingsLib/Three-Phase Transformer (Two Windings)  Winding1Connection=Delta (D1)  Winding2Connection=Yg  CoreType=Three single-phase transformers  SetSaturation=off  Hysteresis=off  DataFile='hysteresis'  SetInitialFlux=off  Measurements=None  UNITS=pu  NominalPower=[ 1000e6 60 ]  Winding1="[ 20e3*1.0  1e-6  0]"  Winding2="[ 345e3*taps(10)  1e-6  0.0181*s]"  Rm=500  Lm=500  L0=0.49998  Saturation="[ 0,0  ;  0.005,1.2  ;  1.0,1.4 ]"  InitialFluxes=[ 0.8 , -0.8 , 0.7 ]  BreakLoop=off  DiscreteSolver=Trapezoidal iterative  DataType=off  TransfoNumber=0
  T2: 900MVA 20 kV/230 kV3 : spsThreePhaseTransformerTwoWindingsLib/Three-Phase Transformer (Two Windings)  Winding1Connection=Delta (D1)  Winding2Connection=Yg  CoreType=Three single-phase transformers  SetSaturation=off  Hysteresis=off  DataFile='hysteresis'  SetInitialFlux=off  Measurements=None  UNITS=pu  NominalPower=[ 1000e6 60 ]  Winding1="[ 20e3*1.0 1e-6  0]"  Winding2="[ 345e3*taps(2)  1e-6  0.0250*s ]"  Rm=500  Lm=500  L0=0.5  Saturation="[ 0,0  ;  0.005,1.2  ;  1.0,1.4 ]"  InitialFluxes=[ 0.8 , -0.8 , 0.7 ]  BreakLoop=off  DiscreteSolver=Trapezoidal iterative  DataType=off  TransfoNumber=0
  T2: 900MVA 20 kV/230 kV4 : spsThreePhaseTransformerTwoWindingsLib/Three-Phase Transformer (Two Windings)  Winding1Connection=Y  Winding2Connection=Y  CoreType=Three single-phase transformers  SetSaturation=off  Hysteresis=off  DataFile='hysteresis'  SetInitialFlux=off  Measurements=None  UNITS=pu  NominalPower=[ 1000e6 60 ]  Winding1="[ 345e3 .0008*s  0]"  Winding2="[ 230e3*1.00  .0008*s   .0435*s]"  Rm=500  Lm=500  L0=0.5  Saturation="[ 0,0  ;  0.005,1.2  ;  1.0,1.4 ]"  InitialFluxes=[ 0.8 , -0.8 , 0.7 ]  BreakLoop=off  DiscreteSolver=Trapezoidal iterative  DataType=off  TransfoNumber=0
  T2: 900MVA 20 kV/230 kV5 : spsThreePhaseTransformerTwoWindingsLib/Three-Phase Transformer (Two Windings)  Winding1Connection=Y  Winding2Connection=Y  CoreType=Three single-phase transformers  SetSaturation=off  Hysteresis=off  DataFile='hysteresis'  SetInitialFlux=off  Measurements=None  UNITS=pu  NominalPower=[ 1000e6 60 ]  Winding1="[ 345e3 .0008*s  0]"  Winding2="[ 230e3*1.00 .0008*s  .0435*s]"  Rm=500  Lm=500  L0=0.5  Saturation="[ 0,0  ;  0.005,1.2  ;  1.0,1.4 ]"  InitialFluxes=[ 0.8 , -0.8 , 0.7 ]  BreakLoop=off  DiscreteSolver=Trapezoidal iterative  DataType=off  TransfoNumber=0
  T2: 900MVA 20 kV/230 kV6 : spsThreePhaseTransformerTwoWindingsLib/Three-Phase Transformer (Two Windings)  Winding1Connection=Delta (D1)  Winding2Connection=Yg  CoreType=Three single-phase transformers  SetSaturation=off  Hysteresis=off  DataFile='hysteresis'  SetInitialFlux=off  Measurements=None  UNITS=pu  NominalPower=[ 1000e6 60 ]  Winding1="[ 20e3*1.0 1e-6  0]"  Winding2="[ 345e3*taps(3)  1e-6    0.020*s*1.0 ]"  Rm=500  Lm=500  L0=0.5  Saturation="[ 0,0  ;  0.005,1.2  ;  1.0,1.4 ]"  InitialFluxes=[ 0.8 , -0.8 , 0.7 ]  BreakLoop=off  DiscreteSolver=Trapezoidal iterative  DataType=off  TransfoNumber=0
  T2: 900MVA 20 kV/230 kV7 : spsThreePhaseTransformerTwoWindingsLib/Three-Phase Transformer (Two Windings)  Winding1Connection=Delta (D1)  Winding2Connection=Yg  CoreType=Three single-phase transformers  SetSaturation=off  Hysteresis=off  DataFile='hysteresis'  SetInitialFlux=off  Measurements=None  UNITS=pu  NominalPower=[ 1000e6 60 ]  Winding1="[ 20e3*1.  0.0004*s  0]"  Winding2="[ 345e3*taps(9)  0.0004*s  0.0156*s]"  Rm=500  Lm=500  L0=0.5  Saturation="[ 0,0  ;  0.005,1.2  ;  1.0,1.4 ]"  InitialFluxes=[ 0.8 , -0.8 , 0.7 ]  BreakLoop=off  DiscreteSolver=Trapezoidal iterative  DataType=off  TransfoNumber=0
  T2: 900MVA 20 kV/230 kV8 : spsThreePhaseTransformerTwoWindingsLib/Three-Phase Transformer (Two Windings)  Winding1Connection=Y  Winding2Connection=Y  CoreType=Three single-phase transformers  SetSaturation=off  Hysteresis=off  DataFile='hysteresis'  SetInitialFlux=off  Measurements=None  UNITS=pu  NominalPower=[ 1000e6 60 ]  Winding1="[ 345e3*1.0  0.00035*s   0]"  Winding2="[ 345e3*1.00 0.00035*s  0.0138*s]"  Rm=500  Lm=500  L0=0.5  Saturation="[ 0,0  ;  0.005,1.2  ;  1.0,1.4 ]"  InitialFluxes=[ 0.8 , -0.8 , 0.7 ]  BreakLoop=off  DiscreteSolver=Trapezoidal iterative  DataType=off  TransfoNumber=0
  T2: 900MVA 20 kV/230 kV9 : spsThreePhaseTransformerTwoWindingsLib/Three-Phase Transformer (Two Windings)  Winding1Connection=Delta (D1)  Winding2Connection=Yg  CoreType=Three single-phase transformers  SetSaturation=off  Hysteresis=off  DataFile='hysteresis'  SetInitialFlux=off  Measurements=None  UNITS=pu  NominalPower=[ 1000e6 60 ]  Winding1="[ 20e3*1.00 0.00045*s  0]"  Winding2="[ 345e3*taps(5)  0.00045*s  0.0180*s]"  Rm=500  Lm=500  L0=0.5  Saturation="[ 0,0  ;  0.005,1.2  ;  1.0,1.4 ]"  InitialFluxes=[ 0.8 , -0.8 , 0.7 ]  BreakLoop=off  DiscreteSolver=Trapezoidal iterative  DataType=off  TransfoNumber=0
  TL<13>-<14> : op_dpl_lib/Distributed Parameters Line  SimulationMode=ARTEMIS model  Phases=3  Frequency=60  Resistance=[1.071 4.285]/TL_13_14_len  Inductance="[0.032  0.095]/TL_13_14_len"  Capacitance=[0.384e-6 0.175e-6]/TL_13_14_len  Length=TL_13_14_len  Measurements=None  mask(Artemis Distributed Parameters Line){}
  TL<14>-<15> : op_dpl_lib/Distributed Parameters Line  SimulationMode=ARTEMIS model  Phases=3  Frequency=60  Resistance=[2.142 8.57]/TL_14_15_len  Inductance="[0.069  0.206]/TL_14_15_len"  Capacitance=[0.816e-6 0.371e-6]/TL_14_15_len  Length=TL_14_15_len  Measurements=None
  TL<15>-<16> : op_dpl_lib/Distributed Parameters Line  SimulationMode=ARTEMIS model  Phases=3  Frequency=60  Resistance=[1.071 4.285]/TL_15_16_len  Inductance="[0.03  0.089]/TL_15_16_len"  Capacitance=[0.381e-6 0.173e-6]/TL_15_16_len  Length=TL_15_16_len  Measurements=None
  TL<16>-<17> : op_dpl_lib/Distributed Parameters Line  SimulationMode=ARTEMIS model  Phases=3  Frequency=60  Resistance=[0.8332 3.33]/TL_16_17_len  Inductance="[0.028  0.084]/TL_16_17_len"  Capacitance=[0.299e-6 0.136e-6]/TL_16_17_len  Length=TL_16_17_len  Measurements=None
  TL<16>-<19> : op_dpl_lib/Distributed Parameters Line  SimulationMode=ARTEMIS model  Phases=3  Frequency=60  Resistance=[1.904 7.618]/TL_16_19_len  Inductance="[0.062  0.185]/TL_16_19_len"  Capacitance=[0.677e-6 0.308e-6]/TL_16_19_len  Length=TL_16_19_len  Measurements=None
  TL<16>-<21> : op_dpl_lib/Distributed Parameters Line  SimulationMode=ARTEMIS model  Phases=3  Frequency=60  Resistance=[0.9522 3.809]/TL_16_21_len  Inductance="[0.043  0.128]/TL_16_21_len"  Capacitance=[0.568e-6 0.258e-6]/TL_16_21_len  Length=TL_16_21_len  Measurements=None
  TL<16>-<24> : op_dpl_lib/Distributed Parameters Line  SimulationMode=ARTEMIS model  Phases=3  Frequency=60  Resistance=[0.357 1.428]/TL_16_24_len  Inductance="[0.019  0.056]/TL_16_24_len"  Capacitance=[0.152e-6 0.069e-6]/TL_16_24_len  Length=TL_16_24_len  Measurements=None
  TL<17>-<18> : op_dpl_lib/Distributed Parameters Line  SimulationMode=ARTEMIS model  Phases=3  Frequency=60  Resistance=[0.833 3.333]/TL_17_18_len  Inductance="[0.026  0.078]/TL_17_18_len"  Capacitance=[0.294e-6 0.134e-6]/TL_17_18_len  Length=TL_17_18_len  Measurements=None
  TL<17>-<27> : op_dpl_lib/Distributed Parameters Line  SimulationMode=ARTEMIS model  Phases=3  Frequency=60  Resistance=[1.547 6.189]/TL_17_27_len  Inductance="[0.055  0.164]/TL_17_27_len"  Capacitance=[0.717e-6 0.326e-6]/TL_17_27_len  Length=TL_17_27_len  Measurements=None
  TL<1>-<2> : op_dpl_lib/Distributed Parameters Line  SimulationMode=ARTEMIS model  Phases=3  Frequency=60  Resistance=[4.166 16.66]/TL_1_2_len  Inductance="[0.13  0.389]/TL_1_2_len"  Capacitance=[1.56e-6 0.708e-6]/TL_1_2_len  Length=TL_1_2_len  Measurements=None
  TL<1>-<39> : op_dpl_lib/Distributed Parameters Line  SimulationMode=ARTEMIS model  Phases=3  Frequency=60  Resistance=[1.19 4.76]/TL_1_39_len  Inductance="[0.079  0.237]/TL_1_39_len"  Capacitance=[1.67e-6 0.7599e-6]/TL_1_39_len  Length=TL_1_39_len  Measurements=None
  TL<21>-<22> : op_dpl_lib/Distributed Parameters Line  SimulationMode=ARTEMIS model  Phases=3  Frequency=60  Resistance=[0.9522 3.809]/TL_21_22_len  Inductance="[0.044  0.133]/TL_21_22_len"  Capacitance=[0.572e-6 0.26e-6]/TL_21_22_len  Length=TL_21_22_len  Measurements=None
  TL<22>-<23> : op_dpl_lib/Distributed Parameters Line  SimulationMode=ARTEMIS model  Phases=3  Frequency=60  Resistance=[0.714 2.857]/TL_22_23_len  Inductance="[0.03  0.091]/TL_22_23_len"  Capacitance=[0.411e-6 0.187e-6]/TL_22_23_len  Length=TL_22_23_len  Measurements=None
  TL<24>-<23> : op_dpl_lib/Distributed Parameters Line  SimulationMode=ARTEMIS model  Phases=3  Frequency=60  Resistance=[2.619 10.474]/TL_24_23_len  Inductance="[0.111  0.332]/TL_24_23_len"  Capacitance=[0.805e-6 0.365e-6]/TL_24_23_len  Length=TL_24_23_len  Measurements=None
  TL<25>-<26> : op_dpl_lib/Distributed Parameters Line  SimulationMode=ARTEMIS model  Phases=3  Frequency=60  Resistance=[3.809 15.235]/TL_25_26_len  Inductance="[0.102  0.306]/TL_25_26_len"  Capacitance=[1.143e-6 0.52e-6]/TL_25_26_len  Length=TL_25_26_len  Measurements=None
  TL<26>--<27> : op_dpl_lib/Distributed Parameters Line  SimulationMode=ARTEMIS model  Phases=3  Frequency=60  Resistance=[1.666 6.665]/TL_26_27_len  Inductance="[0.046  0.139]/TL_26_27_len"  Capacitance=[0.534e-6 0.243e-6]/TL_26_27_len  Length=TL_26_27_len  Measurements=None
  TL<26>-<28> : op_dpl_lib/Distributed Parameters Line  SimulationMode=ARTEMIS model  Phases=3  Frequency=60  Resistance=[5.118 20.472]/TL_26_28_len  Inductance="[0.15  0.449]/TL_26_28_len"  Capacitance=[1.739e-6 0.791e-6]/TL_26_28_len  Length=TL_26_28_len  Measurements=None
  TL<26>-<28>1 : op_dpl_lib/Distributed Parameters Line  SimulationMode=ARTEMIS model  Phases=3  Frequency=60  Resistance=[5.118 20.472]/TL_26_28_len  Inductance="[0.15  0.449]/TL_26_28_len"  Capacitance=[1.739e-6 0.791e-6]/TL_26_28_len  Length=TL_26_28_len  Measurements=None
  TL<26>-<28>2 : op_dpl_lib/Distributed Parameters Line  SimulationMode=ARTEMIS model  Phases=3  Frequency=60  Resistance=[5.118 20.472]/TL_26_28_len  Inductance="[0.15  0.449]/TL_26_28_len"  Capacitance=[1.739e-6 0.791e-6]/TL_26_28_len  Length=TL_26_28_len  Measurements=None
  TL<26>-<29> : op_dpl_lib/Distributed Parameters Line  SimulationMode=ARTEMIS model  Phases=3  Frequency=60  Resistance=[6.784 27.138]/TL_26_29_len  Inductance="[0.197  0.592]/TL_26_29_len"  Capacitance=[2.293e-6 1.043e-6]/TL_26_29_len  Length=TL_26_29_len  Measurements=None
  TL<28>-<29> : op_dpl_lib/Distributed Parameters Line  SimulationMode=ARTEMIS model  Phases=3  Frequency=60  Resistance=[1.666 6.665]/TL_28_29_len  Inductance="[0.048  0.143]/TL_28_29_len"  Capacitance=[0.555e-6 0.252e-6]/TL_28_29_len  Length=TL_28_29_len  Measurements=None
  TL<2>-<25> : op_dpl_lib/Distributed Parameters Line  SimulationMode=ARTEMIS model  Phases=3  Frequency=60  Resistance=[8.33 33.3]/TL_2_25_len  Inductance="[0.027  0.082]/TL_2_25_len"  Capacitance=[0.325e-6 0.148e-6]/TL_2_25_len  Length=TL_2_25_len  Measurements=None
  TL<2>-<3> : op_dpl_lib/Distributed Parameters Line  SimulationMode=ARTEMIS model  Phases=3  Frequency=60  Resistance=[1.547 6.189]/TL_2_2_len  Inductance="[0.048  0.143]/TL_2_2_len"  Capacitance=[0.573e-6 0.261e-6]/TL_2_2_len  Length=TL_2_2_len  Measurements=None
  TL<2>-<3>1 : op_dpl_lib/Distributed Parameters Line  SimulationMode=ARTEMIS model  Phases=3  Frequency=60  Resistance=[1.547 6.189]/TL_2_2_len  Inductance="[0.048  0.143]/TL_2_2_len"  Capacitance=[0.573e-6 0.261e-6]/TL_2_2_len  Length=TL_2_2_len  Measurements=None
  TL<3>-<18> : op_dpl_lib/Distributed Parameters Line  SimulationMode=ARTEMIS model  Phases=3  Frequency=60  Resistance=[1.309 5.237]/TL_3_18_len  Inductance="[0.042  0.126]/TL_3_18_len"  Capacitance=[0.476e-6 0.217e-6]/TL_3_18_len  Length=TL_3_18_len  Measurements=None
  TL<3>-<4> : op_dpl_lib/Distributed Parameters Line  SimulationMode=ARTEMIS model  Phases=3  Frequency=60  Resistance=[1.547 6.18]/TL_3_4_len  Inductance="[0.067  0.208]/TL_3_4_len"  Capacitance=[0.493e-6 0.224e-6]/TL_3_4_len  Length=TL_3_4_len*100  Measurements=None
  TL<3>-<4>1 : op_dpl_lib/Distributed Parameters Line  SimulationMode=ARTEMIS model  Phases=3  Frequency=60  Resistance=[1.547 6.18]/TL_3_4_len  Inductance="[0.067  0.208]/TL_3_4_len"  Capacitance=[0.493e-6 0.224e-6]/TL_3_4_len  Length=TL_3_4_len*100  Measurements=None
  TL<3>-<4>2 : op_dpl_lib/Distributed Parameters Line  SimulationMode=ARTEMIS model  Phases=3  Frequency=60  Resistance=[1.547 6.18]/TL_3_4_len  Inductance="[0.067  0.208]/TL_3_4_len"  Capacitance=[0.493e-6 0.224e-6]/TL_3_4_len  Length=TL_3_4_len  Measurements=None
  TL<3>-<4>3 : op_dpl_lib/Distributed Parameters Line  SimulationMode=ARTEMIS model  Phases=3  Frequency=60  Resistance=[1.547 6.18]/TL_3_4_len  Inductance="[0.067  0.208]/TL_3_4_len"  Capacitance=[0.493e-6 0.224e-6]/TL_3_4_len  Length=TL_3_4_len  Measurements=None
  TL<4>-<14> : op_dpl_lib/Distributed Parameters Line  SimulationMode=ARTEMIS model  Phases=3  Frequency=60  Resistance=[0.9522 3.808]/TL_4_14_len  Inductance="[0.041  0.1223]/TL_4_14_len"  Capacitance=[0.308e-6 0.14e-6]/TL_4_14_len  Length=TL_4_14_len  Measurements=None
  TL<4>-<5> : op_dpl_lib/Distributed Parameters Line  SimulationMode=ARTEMIS model  Phases=3  Frequency=60  Resistance=[0.952 3.809]/TL_4_5_len  Inductance="[0.04  0.121]/TL_4_5_len"  Capacitance=[0.299e-6 0.136e-6]/TL_4_5_len  Length=TL_4_5_len  Measurements=None
  TL<5>-<8> : op_dpl_lib/Distributed Parameters Line  SimulationMode=ARTEMIS model  Phases=3  Frequency=60  Resistance=[0.952 3.809]/TL_5_8_len  Inductance="[0.035  0.106]/TL_5_8_len"  Capacitance=[0.329e-6 0.15e-6]/TL_5_8_len  Length=TL_5_8_len  Measurements=None
  TL<6>-<11> : op_dpl_lib/Distributed Parameters Line  SimulationMode=ARTEMIS model  Phases=3  Frequency=60  Resistance=[0.833 3.333]/TL_6_11_len  Inductance="[0.026  0.078]/TL_6_11_len"  Capacitance=[0.31e-6 0.141e-6]/TL_6_11_len  Length=TL_6_11_len  Measurements=None
  TL<6>-<7> : op_dpl_lib/Distributed Parameters Line  SimulationMode=ARTEMIS model  Phases=3  Frequency=60  Resistance=[0.714 2.857]/TL_6_7_len  Inductance="[0.029  0.087]/TL_6_7_len"  Capacitance=[0.252e-6 0.114e-6]/TL_6_7_len  Length=TL_6_7_len  Measurements=None
  TL<8>-<9> : op_dpl_lib/Distributed Parameters Line  SimulationMode=ARTEMIS model  Phases=3  Frequency=60  Resistance=[2.738 10.95]/TL_8_9_len  Inductance="[0.115  0.344]/TL_8_9_len"  Capacitance=[0.848e-6 0.385e-6]/TL_8_9_len  Length=TL_8_9_len  Measurements=None
  TL<9>-<39> : op_dpl_lib/Distributed Parameters Line  SimulationMode=ARTEMIS model  Phases=3  Frequency=60  Resistance=[1.19 4.761]/TL_9_39_len  Inductance="[0.079  0.237]/TL_9_39_len"  Capacitance=[2.674e-6 1.216e-6]/TL_9_39_len  Length=TL_9_39_len  Measurements=None
  Terminator{1..10} (10 alike) : Terminator
  Terminator15 : Terminator  Commented=on
  Three-Phase V-I Measurement1 : spsThreePhaseVIMeasurementLib/Three-Phase V-I Measurement  VoltageMeasurement=phase-to-ground  SetLabelV=off  LabelV=Vabc  Vpu=off  VpuLL=off  CurrentMeasurement=yes  SetLabelI=off  LabelI=Iabc  Ipu=off  Pbase=100e6  Vbase=500e3  OutputType=Complex  PhasorSimulation=off  PSBequivalent=0
  Three-Phase Breaker : spsThreePhaseBreakerLib/Three-Phase Breaker  InitialState=closed  SwitchA=on  SwitchB=on  SwitchC=on  SwitchTimes="[3  500]"  External=off  BreakerResistance=0.01  SnubberResistance=1e6  SnubberCapacitance=inf  Measurements=None
  dummy D-Y xfo 20kV/345kV : spsThreePhaseTransformerTwoWindingsLib/Three-Phase Transformer (Two Windings)  Winding1Connection=Delta (D1)  Winding2Connection=Yg  CoreType=Three single-phase transformers  SetSaturation=off  Hysteresis=off  DataFile='hysteresis'  SetInitialFlux=off  Measurements=None  UNITS=pu  NominalPower=[ 1000e6 60 ]  Winding1=[20e3 1e-02 0]  Winding2=[345e3 1e-06 0.00001]  Rm=500  Lm=500.01  L0=0.5  Saturation=[0 0;0.0050001 1.2;0.99998 1.4]  InitialFluxes=[0.8 -0.8 0.7]  BreakLoop=off  DiscreteSolver=Trapezoidal iterative  DataType=off  TransfoNumber=0
  load12 : spsThreePhaseParallelRLCLoadLib/Three-Phase Parallel RLC Load  LConnTagsString=A|B|C  Configuration=Y (grounded)  NominalVoltage=(216114)*0.999402  Vabc=[1e3 1e3 1e3]  Vabcp=[1e3 1e3 1e3]  NominalFrequency=60  UnbalancedPower=off  ActivePower=7.5e6  InductivePower=88e6  CapacitivePower=0  Pabc=[10e3 9e3 11e3]  QLabc=[100 90 110]  QCabc=[100 90 110]  Pabcp=[10e3 9e3 11e3]  QLabcp=[100 90 110]  QCabcp=[100 90 110]  Measurements=None  LoadType=constant PQ
  load15 : spsThreePhaseParallelRLCLoadLib/Three-Phase Parallel RLC Load  LConnTagsString=A|B|C  Configuration=Y (grounded)  NominalVoltage=(334507)*0.99961  Vabc=[1e3 1e3 1e3]  Vabcp=[1e3 1e3 1e3]  NominalFrequency=60  UnbalancedPower=off  ActivePower=320e6  InductivePower=153e6  CapacitivePower=0  Pabc=[10e3 9e3 11e3]  QLabc=[100 90 110]  QCabc=[100 90 110]  Pabcp=[10e3 9e3 11e3]  QLabcp=[100 90 110]  QCabcp=[100 90 110]  Measurements=None  LoadType=constant PQ
  load16 : spsThreePhaseParallelRLCLoadLib/Three-Phase Parallel RLC Load  LConnTagsString=A|B|C  Configuration=Y (grounded)  NominalVoltage=(341094)*0.999749  Vabc=[1e3 1e3 1e3]  Vabcp=[1e3 1e3 1e3]  NominalFrequency=60  UnbalancedPower=off  ActivePower=329e6  InductivePower=32.3e6  CapacitivePower=0  Pabc=[10e3 9e3 11e3]  QLabc=[100 90 110]  QCabc=[100 90 110]  Pabcp=[10e3 9e3 11e3]  QLabcp=[100 90 110]  QCabcp=[100 90 110]  Measurements=None  LoadType=constant PQ
  load18 : spsThreePhaseParallelRLCLoadLib/Three-Phase Parallel RLC Load  LConnTagsString=A|B|C  Configuration=Y (grounded)  NominalVoltage=(341941)*0.999662  Vabc=[1e3 1e3 1e3]  Vabcp=[1e3 1e3 1e3]  NominalFrequency=60  UnbalancedPower=off  ActivePower=158e6  InductivePower=30e6  CapacitivePower=0  Pabc=[10e3 9e3 11e3]  QLabc=[100 90 110]  QCabc=[100 90 110]  Pabcp=[10e3 9e3 11e3]  QLabcp=[100 90 110]  QCabcp=[100 90 110]  Measurements=None  LoadType=constant PQ
  load2 : spsThreePhaseParallelRLCLoadLib/Three-Phase Parallel RLC Load  Commented=on  LConnTagsString=A|B|C  Configuration=Y (grounded)  NominalVoltage=(351683)*0.999933  Vabc=[1e3 1e3 1e3]  Vabcp=[1e3 1e3 1e3]  NominalFrequency=60  UnbalancedPower=off  ActivePower=5e6  InductivePower=27.6e6  CapacitivePower=0  Pabc=[10e3 9e3 11e3]  QLabc=[100 90 110]  QCabc=[100 90 110]  Pabcp=[10e3 9e3 11e3]  QLabcp=[100 90 110]  QCabcp=[100 90 110]  Measurements=None  LoadType=constant PQ
  load20 : spsThreePhaseParallelRLCLoadLib/Three-Phase Parallel RLC Load  LConnTagsString=A|B|C  Configuration=Y (grounded)  NominalVoltage=(340545)*0.999951  Vabc=[1e3 1e3 1e3]  Vabcp=[1e3 1e3 1e3]  NominalFrequency=60  UnbalancedPower=off  ActivePower=628e6  InductivePower=103e6  CapacitivePower=0  Pabc=[10e3 9e3 11e3]  QLabc=[100 90 110]  QCabc=[100 90 110]  Pabcp=[10e3 9e3 11e3]  QLabcp=[100 90 110]  QCabcp=[100 90 110]  Measurements=None  LoadType=constant PQ
  load21 : spsThreePhaseParallelRLCLoadLib/Three-Phase Parallel RLC Load  LConnTagsString=A|B|C  Configuration=Y (grounded)  NominalVoltage=(343449)*0.999826  Vabc=[1e3 1e3 1e3]  Vabcp=[1e3 1e3 1e3]  NominalFrequency=60  UnbalancedPower=off  ActivePower=274e6  InductivePower=115e6  CapacitivePower=0  Pabc=[10e3 9e3 11e3]  QLabc=[100 90 110]  QCabc=[100 90 110]  Pabcp=[10e3 9e3 11e3]  QLabcp=[100 90 110]  QCabcp=[100 90 110]  Measurements=None  LoadType=constant PQ
  load23 : spsThreePhaseParallelRLCLoadLib/Three-Phase Parallel RLC Load  LConnTagsString=A|B|C  Configuration=Y (grounded)  NominalVoltage=(352041)*0.99991  Vabc=[1e3 1e3 1e3]  Vabcp=[1e3 1e3 1e3]  NominalFrequency=60  UnbalancedPower=off  ActivePower=247.5e6  InductivePower=84.6e6  CapacitivePower=0  Pabc=[10e3 9e3 11e3]  QLabc=[100 90 110]  QCabc=[100 90 110]  Pabcp=[10e3 9e3 11e3]  QLabcp=[100 90 110]  QCabcp=[100 90 110]  Measurements=None  LoadType=constant PQ
  load24 : spsThreePhaseParallelRLCLoadLib/Three-Phase Parallel RLC Load  LConnTagsString=A|B|C  Configuration=Y (grounded)  NominalVoltage=(343942)*0.999774  Vabc=[1e3 1e3 1e3]  Vabcp=[1e3 1e3 1e3]  NominalFrequency=60  UnbalancedPower=off  ActivePower=308.6e6  InductivePower=0  CapacitivePower=92e6  Pabc=[10e3 9e3 11e3]  QLabc=[100 90 110]  QCabc=[100 90 110]  Pabcp=[10e3 9e3 11e3]  QLabcp=[100 90 110]  QCabcp=[100 90 110]  Measurements=None  LoadType=constant PQ
  load25 : spsThreePhaseParallelRLCLoadLib/Three-Phase Parallel RLC Load  LConnTagsString=A|B|C  Configuration=Y (grounded)  NominalVoltage=(354798)*0.99991  Vabc=[1e3 1e3 1e3]  Vabcp=[1e3 1e3 1e3]  NominalFrequency=60  UnbalancedPower=off  ActivePower=224e6  InductivePower=47.2e6  CapacitivePower=0  Pabc=[10e3 9e3 11e3]  QLabc=[100 90 110]  QCabc=[100 90 110]  Pabcp=[10e3 9e3 11e3]  QLabcp=[100 90 110]  QCabcp=[100 90 110]  Measurements=None  LoadType=constant PQ
  load26 : spsThreePhaseParallelRLCLoadLib/Three-Phase Parallel RLC Load  LConnTagsString=A|B|C  Configuration=Y (grounded)  NominalVoltage=(351241)*0.999873  Vabc=[1e3 1e3 1e3]  Vabcp=[1e3 1e3 1e3]  NominalFrequency=60  UnbalancedPower=off  ActivePower=139e6  InductivePower=17e6  CapacitivePower=0  Pabc=[10e3 9e3 11e3]  QLabc=[100 90 110]  QCabc=[100 90 110]  Pabcp=[10e3 9e3 11e3]  QLabcp=[100 90 110]  QCabcp=[100 90 110]  Measurements=None  LoadType=constant PQ
  load27 : spsThreePhaseParallelRLCLoadLib/Three-Phase Parallel RLC Load  LConnTagsString=A|B|C  Configuration=Y (grounded)  NominalVoltage=(345100)*0.999809  Vabc=[1e3 1e3 1e3]  Vabcp=[1e3 1e3 1e3]  NominalFrequency=60  UnbalancedPower=off  ActivePower=281e6  InductivePower=75.5e6  CapacitivePower=0  Pabc=[10e3 9e3 11e3]  QLabc=[100 90 110]  QCabc=[100 90 110]  Pabcp=[10e3 9e3 11e3]  QLabcp=[100 90 110]  QCabcp=[100 90 110]  Measurements=None  LoadType=constant PQ
  load28 : spsThreePhaseParallelRLCLoadLib/Three-Phase Parallel RLC Load  LConnTagsString=A|B|C  Configuration=Y (grounded)  NominalVoltage=(351683)*0.999933  Vabc=[1e3 1e3 1e3]  Vabcp=[1e3 1e3 1e3]  NominalFrequency=60  UnbalancedPower=off  ActivePower=206e6  InductivePower=27.6e6  CapacitivePower=0  Pabc=[10e3 9e3 11e3]  QLabc=[100 90 110]  QCabc=[100 90 110]  Pabcp=[10e3 9e3 11e3]  QLabcp=[100 90 110]  QCabcp=[100 90 110]  Measurements=None  LoadType=constant PQ
  load29 : spsThreePhaseParallelRLCLoadLib/Three-Phase Parallel RLC Load  LConnTagsString=A|B|C  Configuration=Y (grounded)  NominalVoltage=(352166)*0.999961  Vabc=[1e3 1e3 1e3]  Vabcp=[1e3 1e3 1e3]  NominalFrequency=60  UnbalancedPower=off  ActivePower=283.5e6  InductivePower=26.9e6  CapacitivePower=0  Pabc=[10e3 9e3 11e3]  QLabc=[100 90 110]  QCabc=[100 90 110]  Pabcp=[10e3 9e3 11e3]  QLabcp=[100 90 110]  QCabcp=[100 90 110]  Measurements=None  LoadType=constant PQ
  load3 : spsThreePhaseParallelRLCLoadLib/Three-Phase Parallel RLC Load  LConnTagsString=A|B|C  Configuration=Y (grounded)  NominalVoltage=(345000)  Vabc=[1e3 1e3 1e3]  Vabcp=[1e3 1e3 1e3]  NominalFrequency=60  UnbalancedPower=off  ActivePower=322e6  InductivePower=2.4e6  CapacitivePower=0  Pabc=[10e3 9e3 11e3]  QLabc=[100 90 110]  QCabc=[100 90 110]  Pabcp=[10e3 9e3 11e3]  QLabcp=[100 90 110]  QCabcp=[100 90 110]  Measurements=None  LoadType=constant PQ
  load31 : spsThreePhaseParallelRLCLoadLib/Three-Phase Parallel RLC Load  LConnTagsString=A|B|C  Configuration=Y (grounded)  NominalVoltage=(22000)*0.982  Vabc=[1e3 1e3 1e3]  Vabcp=[1e3 1e3 1e3]  NominalFrequency=60  UnbalancedPower=off  ActivePower=9.2e6  InductivePower=4.6e6  CapacitivePower=0  Pabc=[10e3 9e3 11e3]  QLabc=[100 90 110]  QCabc=[100 90 110]  Pabcp=[10e3 9e3 11e3]  QLabcp=[100 90 110]  QCabcp=[100 90 110]  Measurements=None  LoadType=constant PQ
  load39 : spsThreePhaseParallelRLCLoadLib/Three-Phase Parallel RLC Load  LConnTagsString=A|B|C  Configuration=Y (grounded)  NominalVoltage=(345000)*1.03  Vabc=[1e3 1e3 1e3]  Vabcp=[1e3 1e3 1e3]  NominalFrequency=60  UnbalancedPower=off  ActivePower=1104e6  InductivePower=250e6  CapacitivePower=0  Pabc=[10e3 9e3 11e3]  QLabc=[100 90 110]  QCabc=[100 90 110]  Pabcp=[10e3 9e3 11e3]  QLabcp=[100 90 110]  QCabcp=[100 90 110]  Measurements=None  LoadType=constant PQ
  load4 : spsThreePhaseParallelRLCLoadLib/Three-Phase Parallel RLC Load  LConnTagsString=A|B|C  Configuration=Y (grounded)  NominalVoltage=(329948)*0.999007  Vabc=[1e3 1e3 1e3]  Vabcp=[1e3 1e3 1e3]  NominalFrequency=60  UnbalancedPower=off  ActivePower=500e6  InductivePower=184e6  CapacitivePower=0  Pabc=[10e3 9e3 11e3]  QLabc=[100 90 110]  QCabc=[100 90 110]  Pabcp=[10e3 9e3 11e3]  QLabcp=[100 90 110]  QCabcp=[100 90 110]  Measurements=None  LoadType=constant PQ
  load7 : spsThreePhaseParallelRLCLoadLib/Three-Phase Parallel RLC Load  LConnTagsString=A|B|C  Configuration=Y (grounded)  NominalVoltage=(329980)*0.991241  Vabc=[1e3 1e3 1e3]  Vabcp=[1e3 1e3 1e3]  NominalFrequency=60  UnbalancedPower=off  ActivePower=233e6  InductivePower=84e6  CapacitivePower=0  Pabc=[10e3 9e3 11e3]  QLabc=[100 90 110]  QCabc=[100 90 110]  Pabcp=[10e3 9e3 11e3]  QLabcp=[100 90 110]  QCabcp=[100 90 110]  Measurements=None  LoadType=constant PQ
  load8 : spsThreePhaseParallelRLCLoadLib/Three-Phase Parallel RLC Load  LConnTagsString=A|B|C  Configuration=Y (grounded)  NominalVoltage=(329142)*0.994604  Vabc=[1e3 1e3 1e3]  Vabcp=[1e3 1e3 1e3]  NominalFrequency=60  UnbalancedPower=off  ActivePower=522e6  InductivePower=176e6  CapacitivePower=0  Pabc=[10e3 9e3 11e3]  QLabc=[100 90 110]  QCabc=[100 90 110]  Pabcp=[10e3 9e3 11e3]  QLabcp=[100 90 110]  QCabcp=[100 90 110]  Measurements=None  LoadType=constant PQ
  mag : Outport
  phase : Outport  Port=2
  freq : Outport  Port=3
  peo : Outport  Port=4
  Pg : Outport  Port=5
  mes_WT12 : Outport  Port=6
  mes_WT34 : Outport  Port=7
  wires:
  Three-Phase V-I Measurement1/2 -> Scope1/2
  Three-Phase V-I Measurement1/1 -> Scope1/1
  [Peo10] -> Mux3/10
  [G7_Vmag] -> Mux/7
  Rate Transition1/1 -> PMU_Vpos_60Hz/1(abc)
  PMU_Vpos_60Hz2/1(Mag) -> [G9_Vmag]
  [Peo5] -> Mux3/5
  Mux3/1 -> Memory4/1
  [G3_freq] -> Mux2/3
  [G5_phase] -> Mux1/5
  PMU_Vpos_60Hz6/1(Mag) -> [G5_Vmag]
  Rate Transition10/1 -> PMU_Vpos_60Hz6/1(abc)
  [Peo7] -> Mux3/7
  [Peo3] -> Mux3/3
  PMU_Vpos_60Hz/4(dfdt) -> Terminator1/1
  PMU_Vpos_60Hz6/3(freq) -> [G5_freq]
  PMU_Vpos_60Hz5/3(freq) -> [G3_freq]
  Rate Transition3/1 -> PMU_Vpos_60Hz2/1(abc)
  [Peo8] -> Mux3/8
  Rate Transition6/1 -> PMU_Vpos_60Hz9/1(abc)
  [Peo4] -> Mux3/4
  [Peo1] -> Mux3/1
  PMU_Vpos_60Hz9/3(freq) -> [G7_freq]
  PMU_Vpos_60Hz7/1(Mag) -> [G4_Vmag]
  PMU_Vpos_60Hz8/2(Phase) -> [G6_phase]
  [Peo2] -> Mux3/2
  Rate Transition8/1 -> PMU_Vpos_60Hz7/1(abc)
  PMU_Vpos_60Hz1/4(dfdt) -> Terminator2/1
  PMU_Vpos_60Hz/3(freq) -> [G10_freq]
  [G5_freq] -> Mux2/5
  [Peo6] -> Mux3/6
  [G8_Vmag] -> Mux/8
  Rate Transition13/1 -> Memory3/1
  Rate Transition12/1 -> Memory2/1
  PMU_Vpos_60Hz3/2(Phase) -> [G1_phase]
  Mux2/1 -> Rate Transition13/1, Scope3/1
  PMU_Vpos_60Hz4/2(Phase) -> [G2_phase]
  Mux1/1 -> Rate Transition12/1, Scope2/1
  [G1_phase] -> Mux1/1
  Rate Transition11/1 -> Memory1/1
  [G8_freq] -> Mux2/8
  PMU_Vpos_60Hz5/1(Mag) -> [G3_Vmag]
  Rate Transition9/1 -> PMU_Vpos_60Hz5/1(abc)
  PMU_Vpos_60Hz/2(Phase) -> [G10_phase]
  Rate Transition5/1 -> PMU_Vpos_60Hz4/1(abc)
  PMU_Vpos_60Hz7/2(Phase) -> [G4_phase]
  [G4_freq] -> Mux2/4
  PMU_Vpos_60Hz3/1(Mag) -> [G1_Vmag]
  PMU_Vpos_60Hz8/4(dfdt) -> Terminator9/1
  [G7_freq] -> Mux2/7
  Rate Transition4/1 -> PMU_Vpos_60Hz3/1(abc)
  PMU_Vpos_60Hz1/1(Mag) -> [G8_Vmag]
  [G9_phase] -> Mux1/9
  [G9_Vmag] -> Mux/9
  PMU_Vpos_60Hz1/2(Phase) -> [G8_phase]
  [G2_phase] -> Mux1/2
  [G3_phase] -> Mux1/3
  [G7_phase] -> Mux1/7
  PMU_Vpos_60Hz3/4(dfdt) -> Terminator4/1
  [G10_freq] -> Mux2/10
  Mux/1 -> Rate Transition11/1, Scope/1
  [G8_phase] -> Mux1/8
  [G4_Vmag] -> Mux/4
  [G4_phase] -> Mux1/4
  [G5_Vmag] -> Mux/5
  [G2_Vmag] -> Mux/2
  [G3_Vmag] -> Mux/3
  [G9_freq] -> Mux2/9
  PMU_Vpos_60Hz9/2(Phase) -> [G7_phase]
  PMU_Vpos_60Hz8/1(Mag) -> [G6_Vmag]
  PMU_Vpos_60Hz7/3(freq) -> [G4_freq]
  PMU_Vpos_60Hz4/3(freq) -> [G2_freq]
  PMU_Vpos_60Hz6/2(Phase) -> [G5_phase]
  [G1_freq] -> Mux2/1
  PMU_Vpos_60Hz7/4(dfdt) -> Terminator8/1
  PMU_Vpos_60Hz4/1(Mag) -> [G2_Vmag]
  PMU_Vpos_60Hz9/1(Mag) -> [G7_Vmag]
  [G10_phase] -> Mux1/10
  PMU_Vpos_60Hz5/2(Phase) -> [G3_phase]
  [G2_freq] -> Mux2/2
  [G10_Vmag] -> Mux/10
  PMU_Vpos_60Hz6/4(dfdt) -> Terminator7/1
  Rate Transition7/1 -> PMU_Vpos_60Hz8/1(abc)
  PMU_Vpos_60Hz3/3(freq) -> [G1_freq]
  PMU_Vpos_60Hz8/3(freq) -> [G6_freq]
  PMU_Vpos_60Hz4/4(dfdt) -> Terminator5/1
  PMU_Vpos_60Hz5/4(dfdt) -> Terminator6/1
  Rate Transition2/1 -> PMU_Vpos_60Hz1/1(abc)
  PMU_Vpos_60Hz9/4(dfdt) -> Terminator10/1
  [G1_Vmag] -> Mux/1
  PMU_Vpos_60Hz1/3(freq) -> [G8_freq]
  PMU_Vpos_60Hz2/4(dfdt) -> Terminator3/1
  PMU_Vpos_60Hz2/3(freq) -> [G9_freq]
  [G6_Vmag] -> Mux/6
  PMU_Vpos_60Hz/1(Mag) -> [G10_Vmag]
  [G6_phase] -> Mux1/6
  [G6_freq] -> Mux2/6
  PMU_Vpos_60Hz2/2(Phase) -> [G9_phase]
  [Peo9] -> Mux3/9
  Memory4/1 -> peo/1
  Memory3/1 -> freq/1
  Memory2/1 -> phase/1
  Memory1/1 -> mag/1
  Gain/1 -> Rate Transition5/1
  [Vabc_31] -> Gain/1
  Gain1/1 -> Rate Transition4/1
  [Vabc_39] -> Gain1/1
  [Vabc_29] -> Gain2/1
  Gain2/1 -> Rate Transition3/1
  [Vabc_36] -> Gain3/1
  Gain3/1 -> Rate Transition6/1
  Gain4/1 -> Rate Transition7/1
  [Vabc_35] -> Gain4/1
  Gain5/1 -> Rate Transition8/1
  [Vabc_33] -> Gain5/1
  Gain6/1 -> Rate Transition10/1
  [Vabc_34] -> Gain6/1
  Gain7/1 -> Rate Transition9/1
  [Vabc_32] -> Gain7/1
  Gain8/1 -> Rate Transition2/1
  [Vabc_37] -> Gain8/1
  Gain9/1 -> Rate Transition1/1
  [Vabc_30] -> Gain9/1
  Power/1(Pgen) -> Pg/1
  4 WT/1(mes_WT12) -> mes_WT12/1
  4 WT/2(mes_WT34) -> mes_WT34/1
  connections:
  TL<1>-<39>/LConn3 -- 1/RConn3
  T2: 900MVA 20 kV/230 kV10/LConn3 -- 21/RConn3
  TL<2>-<3>/LConn2 -- 2/RConn2 -- TL<1>-<2>/LConn2
  30/RConn1 -- T2: 900MVA 20 kV/230 kV2/LConn1
  36/LConn3 -- TL<24>-<23>/RConn3 -- TL<22>-<23>/RConn3
  T2: 900MVA 20 kV/230 kV9/RConn1 -- load20/LConn1 -- 20/RConn1
  16/LConn1 -- TL<15>-<16>/LConn1 -- TL<16>-<19>/LConn1 -- TL<16>-<21>/LConn1
  TL<26>--<27>/RConn3 -- load27/LConn3 -- 27/LConn3
  T2: 900MVA 20 kV/230 kV10/RConn1 -- TL<16>-<19>/RConn1 -- 19/LConn1
  TL<17>-<27>/RConn1 -- 17/LConn1 -- TL<16>-<17>/RConn1
  32/LConn3 -- T2: 900MVA 20 kV/230 kV6/LConn3
  TL<24>-<23>/LConn3 -- load24/LConn3 -- 33/RConn3
  load21/LConn2 -- TL<21>-<22>/LConn2 -- TL<3>-<4>3/LConn2 -- 23/RConn2
  load31/LConn3 -- 31/RConn3 -- G2/RConn3
  load18/LConn1 -- 18/LConn1
  6/LConn1 -- 5-6 14 km/RConn1 -- TL<6>-<11>/LConn1
  TL<17>-<27>/RConn2 -- 17/LConn2 -- TL<16>-<17>/RConn2
  TL<26>-<29>/LConn3 -- Three-Phase V-I Measurement1/LConn3
  10-11 14 km/LConn3 -- 11/RConn3
  16/RConn1 -- load16/LConn1 -- TL<16>-<24>/LConn1 -- TL<16>-<17>/LConn1
  load7/LConn3 -- 7-8 15 km/LConn3 -- 7/LConn3
  3/LConn2 -- TL<2>-<3>/RConn2 -- TL<3>-<18>/LConn2
  8/LConn1 -- TL<3>-<4>1/RConn1 -- TL<8>-<9>/RConn1 -- 7-8 15 km/RConn1 -- TL<5>-<8>/RConn1
  18/RConn2 -- TL<3>-<18>/RConn2 -- TL<17>-<18>/LConn2
  TL<17>-<27>/RConn3 -- 17/LConn3 -- TL<16>-<17>/RConn3
  TL<26>-<29>/RConn3 -- TL<28>-<29>/RConn3 -- load29/LConn3 -- 29/RConn3
  5/RConn3 -- 5-6 14 km/LConn3 -- TL<5>-<8>/LConn3
  16/RConn2 -- load16/LConn2 -- TL<16>-<24>/LConn2 -- TL<16>-<17>/LConn2
  T2: 900MVA 20 kV/230 kV4/RConn2 -- T2: 900MVA 20 kV/230 kV5/RConn2 -- 12/RConn2
  load28/LConn1 -- 28/LConn1
  load15/LConn1 -- 15/RConn1 -- TL<14>-<15>/LConn1
  34/LConn3 -- T2: 900MVA 20 kV/230 kV9/LConn3
  TL<4>-<14>/LConn1 -- 4/LConn1 -- TL<3>-<4>/RConn1
  load21/LConn3 -- TL<21>-<22>/LConn3 -- TL<3>-<4>3/LConn3 -- 23/RConn3
  TL<2>-<25>/LConn1 -- load25/LConn1 -- 25/RConn1
  13/LConn1 -- TL<13>-<14>/RConn1 -- T2: 900MVA 20 kV/230 kV5/LConn1
  load18/LConn2 -- 18/LConn2
  T2: 900MVA 20 kV/230 kV9/RConn2 -- load20/LConn2 -- 20/RConn2
  29/RConn1 -- load29/LConn1 -- TL<26>-<29>/RConn1 -- TL<28>-<29>/RConn1
  3/LConn1 -- TL<2>-<3>/RConn1 -- TL<3>-<18>/LConn1
  T2: 900MVA 20 kV/230 kV1/RConn3 -- TL<25>-<26>/LConn3 -- 25/LConn3
  26/LConn3 -- load26/LConn3 -- TL<26>-<28>/LConn3 -- Three-Phase V-I Measurement1/RConn3
  T2: 900MVA 20 kV/230 kV12/LConn2 -- 35/LConn2
  TL<1>-<2>/RConn3 -- 1/LConn3
  T2: 900MVA 20 kV/230 kV12/RConn3 -- load23/LConn3 -- 36/RConn3
  TL<3>-<4>1/RConn2 -- TL<8>-<9>/RConn2 -- 8/LConn2 -- 7-8 15 km/RConn2 -- TL<5>-<8>/RConn2
  5/RConn1 -- 5-6 14 km/LConn1 -- TL<5>-<8>/LConn1
  load15/LConn2 -- 15/RConn2 -- TL<14>-<15>/LConn2
  2/RConn1 -- TL<2>-<3>/LConn1 -- TL<1>-<2>/LConn1
  T2: 900MVA 20 kV/230 kV10/RConn3 -- TL<16>-<19>/RConn3 -- 19/LConn3
  T2: 900MVA 20 kV/230 kV10/RConn2 -- TL<16>-<19>/RConn2 -- 19/LConn2
  31/LConn2 -- T2: 900MVA 20 kV/230 kV3/LConn2
  25/RConn2 -- load25/LConn2 -- TL<2>-<25>/LConn2
  10-11 14 km/RConn1 -- 10-13 14 km/RConn1 -- 10/LConn1
  TL<21>-<22>/LConn1 -- load21/LConn1 -- TL<3>-<4>3/LConn1 -- 23/RConn1
  TL<24>-<23>/LConn2 -- load24/LConn2 -- 33/RConn2
  T2: 900MVA 20 kV/230 kV8/LConn1 -- 19/RConn1
  TL<4>-<5>/RConn1 -- 5/LConn1
  TL<9>-<39>/RConn2 -- 9/LConn2
  31/LConn3 -- T2: 900MVA 20 kV/230 kV3/LConn3
  10-11 14 km/RConn2 -- 10-13 14 km/RConn2 -- 10/LConn2
  T2: 900MVA 20 kV/230 kV11/LConn2 -- 35./LConn2
  load18/LConn3 -- 18/LConn3
  26/RConn3 -- TL<25>-<26>/RConn3 -- TL<26>--<27>/LConn3
  Three-Phase V-I Measurement1/RConn2 -- load26/LConn2 -- TL<26>-<28>/LConn2 -- 26/LConn2
  TL<16>-<24>/RConn3 -- 33/LConn3
  T2: 900MVA 20 kV/230 kV6/RConn1 -- 10/RConn1
  10-11 14 km/RConn3 -- 10-13 14 km/RConn3 -- 10/LConn3
  TL<21>-<22>/RConn3 -- 22/LConn3
  TL<16>-<21>/RConn1 -- 23/LConn1
  load28/LConn3 -- 28/LConn3
  3/LConn3 -- TL<2>-<3>/RConn3 -- TL<3>-<18>/LConn3
  TL<4>-<14>/RConn1 -- TL<14>-<15>/RConn1 -- 14/RConn1
  3/RConn2 -- load3/LConn2 -- TL<3>-<4>/LConn2
  TL<16>-<21>/RConn2 -- 23/LConn2
  4/RConn3 -- load4/LConn3 -- TL<4>-<5>/LConn3
  T2: 900MVA 20 kV/230 kV2/RConn1 -- 2/LConn1 -- TL<2>-<25>/RConn1 -- TL<2>-<3>1/RConn1
  TL<9>-<39>/RConn1 -- 9/LConn1
  T2: 900MVA 20 kV/230 kV5/LConn3 -- TL<13>-<14>/RConn3 -- 13/LConn3
  load12/LConn3 -- 12/LConn3
  TL<8>-<9>/LConn3 -- 9/RConn3
  TL<15>-<16>/RConn3 -- 15/LConn3
  T2: 900MVA 20 kV/230 kV3/RConn2 -- TL<6>-<7>/LConn2 -- 6/RConn2
  T2: 900MVA 20 kV/230 kV11/RConn1 -- TL<22>-<23>/LConn1 -- 22/RConn1
  34/LConn1 -- T2: 900MVA 20 kV/230 kV9/LConn1
  dummy D-Y xfo 20kV/345kV/RConn3 -- 39/RConn3
  10-11 14 km/LConn1 -- 11/RConn1
  T2: 900MVA 20 kV/230 kV8/LConn2 -- 19/RConn2
  TL<26>-<29>/LConn2 -- Three-Phase V-I Measurement1/LConn2
  37/RConn1 -- T2: 900MVA 20 kV/230 kV1/LConn1
  29/RConn2 -- load29/LConn2 -- TL<26>-<29>/RConn2 -- TL<28>-<29>/RConn2
  TL<16>-<24>/RConn1 -- 33/LConn1
  TL<4>-<14>/RConn3 -- TL<14>-<15>/RConn3 -- 14/RConn3
  T2: 900MVA 20 kV/230 kV12/LConn3 -- 35/LConn3
  T2: 900MVA 20 kV/230 kV12/RConn1 -- load23/LConn1 -- 36/RConn1
  35./LConn1 -- T2: 900MVA 20 kV/230 kV11/LConn1
  6/LConn3 -- 5-6 14 km/RConn3 -- TL<6>-<11>/LConn3
  load8/LConn2 -- 8/RConn2
  TL<2>-<3>/LConn3 -- TL<1>-<2>/LConn3 -- 2/RConn3
  26/RConn2 -- TL<25>-<26>/RConn2 -- TL<26>--<27>/LConn2
  T2: 900MVA 20 kV/230 kV8/RConn1 -- 20/LConn1
  4/RConn1 -- load4/LConn1 -- TL<4>-<5>/LConn1
  TL<1>-<2>/RConn2 -- 1/LConn2
  TL<16>-<24>/RConn2 -- 33/LConn2
  T2: 900MVA 20 kV/230 kV4/LConn1 -- TL<6>-<11>/RConn1 -- TL<3>-<4>2/LConn1 -- 11/LConn1
  TL<4>-<14>/LConn3 -- TL<3>-<4>/RConn3 -- 4/LConn3
  T2: 900MVA 20 kV/230 kV12/RConn2 -- load23/LConn2 -- 36/RConn2
  load16/LConn3 -- 16/RConn3 -- TL<16>-<17>/LConn3 -- TL<16>-<24>/LConn3
  TL<9>-<39>/RConn3 -- 9/LConn3
  10-13 14 km/LConn3 -- 13/RConn3
  28/RConn2 -- TL<26>-<28>/RConn2 -- TL<28>-<29>/LConn2
  T2: 900MVA 20 kV/230 kV11/LConn3 -- 35./LConn3
  load31/LConn1 -- 31/RConn1 -- G2/RConn1
  T2: 900MVA 20 kV/230 kV10/LConn1 -- 21/RConn1
  TL<21>-<22>/RConn1 -- 22/LConn1
  T2: 900MVA 20 kV/230 kV12/LConn1 -- 35/LConn1
  22/RConn3 -- TL<22>-<23>/LConn3 -- T2: 900MVA 20 kV/230 kV11/RConn3
  load28/LConn2 -- 28/LConn2
  T2: 900MVA 20 kV/230 kV4/RConn3 -- T2: 900MVA 20 kV/230 kV5/RConn3 -- 12/RConn3
  TL<4>-<14>/LConn2 -- TL<3>-<4>/RConn2 -- 4/LConn2
  36/LConn2 -- TL<24>-<23>/RConn2 -- TL<22>-<23>/RConn2
  T2: 900MVA 20 kV/230 kV9/RConn3 -- load20/LConn3 -- 20/RConn3
  18/RConn3 -- TL<3>-<18>/RConn3 -- TL<17>-<18>/LConn3
  TL<16>-<21>/RConn3 -- 23/LConn3
  16/LConn3 -- TL<15>-<16>/LConn3 -- TL<16>-<19>/LConn3 -- TL<16>-<21>/LConn3
  13/LConn2 -- TL<13>-<14>/RConn2 -- T2: 900MVA 20 kV/230 kV5/LConn2
  30/RConn2 -- T2: 900MVA 20 kV/230 kV2/LConn2
  25/LConn2 -- TL<25>-<26>/LConn2 -- T2: 900MVA 20 kV/230 kV1/RConn2
  TL<16>-<19>/LConn2 -- TL<16>-<21>/LConn2 -- TL<15>-<16>/LConn2 -- 16/LConn2
  load7/LConn2 -- 7-8 15 km/LConn2 -- 7/LConn2
  dummy D-Y xfo 20kV/345kV/RConn2 -- 39/RConn2
  T2: 900MVA 20 kV/230 kV4/LConn3 -- TL<3>-<4>2/LConn3 -- TL<6>-<11>/RConn3 -- 11/LConn3
  load3/LConn3 -- TL<3>-<4>/LConn3 -- 3/RConn3
  39/LConn1 -- load39/LConn1 -- TL<9>-<39>/LConn1 -- TL<1>-<39>/RConn1
  TL<8>-<9>/LConn1 -- 9/RConn1
  T2: 900MVA 20 kV/230 kV8/RConn2 -- 20/LConn2
  TL<2>-<25>/LConn3 -- load25/LConn3 -- 25/RConn3
  T2: 900MVA 20 kV/230 kV8/RConn3 -- 20/LConn3
  39/LConn2 -- load39/LConn2 -- TL<9>-<39>/LConn2 -- TL<1>-<39>/RConn2
  TL<26>--<27>/RConn1 -- load27/LConn1 -- 27/LConn1
  34/LConn2 -- T2: 900MVA 20 kV/230 kV9/LConn2
  TL<15>-<16>/RConn2 -- 15/LConn2
  TL<4>-<5>/RConn2 -- 5/LConn2
  TL<26>-<29>/LConn1 -- Three-Phase V-I Measurement1/LConn1
  load15/LConn3 -- TL<14>-<15>/LConn3 -- 15/RConn3
  TL<8>-<9>/LConn2 -- 9/RConn2
  10/RConn2 -- T2: 900MVA 20 kV/230 kV6/RConn2
  TL<13>-<14>/LConn3 -- 14/LConn3
  5/RConn2 -- 5-6 14 km/LConn2 -- TL<5>-<8>/LConn2
  T2: 900MVA 20 kV/230 kV6/RConn3 -- 10/RConn3
  TL<24>-<23>/LConn1 -- load24/LConn1 -- 33/RConn1
  Three-Phase V-I Measurement1/RConn1 -- load26/LConn1 -- TL<26>-<28>/LConn1 -- 26/LConn1
  TL<6>-<7>/RConn3 -- 7/RConn3
  TL<13>-<14>/LConn1 -- 14/LConn1
  TL<4>-<14>/RConn2 -- TL<14>-<15>/RConn2 -- 14/RConn2
  39/LConn3 -- load39/LConn3 -- TL<9>-<39>/LConn3 -- TL<1>-<39>/RConn3
  37/RConn2 -- T2: 900MVA 20 kV/230 kV1/LConn2
  10-13 14 km/LConn2 -- 13/RConn2
  TL<6>-<7>/RConn2 -- 7/RConn2
  TL<4>-<5>/LConn2 -- load4/LConn2 -- 4/RConn2
  load7/LConn1 -- 7-8 15 km/LConn1 -- 7/LConn1
  load12/LConn1 -- 12/LConn1
  10-13 14 km/LConn1 -- 13/RConn1
  6/RConn3 -- TL<6>-<7>/LConn3 -- T2: 900MVA 20 kV/230 kV3/RConn3
  TL<3>-<4>1/RConn3 -- TL<8>-<9>/RConn3 -- 8/LConn3 -- 7-8 15 km/RConn3 -- TL<5>-<8>/RConn3
  load8/LConn1 -- 8/RConn1
  T2: 900MVA 20 kV/230 kV4/RConn1 -- T2: 900MVA 20 kV/230 kV5/RConn1 -- 12/RConn1
  32/LConn1 -- T2: 900MVA 20 kV/230 kV6/LConn1
  TL<17>-<27>/LConn1 -- 27/RConn1
  T2: 900MVA 20 kV/230 kV3/RConn1 -- TL<6>-<7>/LConn1 -- 6/RConn1
  T2: 900MVA 20 kV/230 kV7/LConn1 -- 38/LConn1
  TL<1>-<39>/LConn1 -- 1/RConn1
  T2: 900MVA 20 kV/230 kV2/RConn3 -- TL<2>-<25>/RConn3 -- 2/LConn3 -- TL<2>-<3>1/RConn3
  30/RConn3 -- T2: 900MVA 20 kV/230 kV2/LConn3
  28/RConn1 -- TL<26>-<28>/RConn1 -- TL<28>-<29>/LConn1
  load8/LConn3 -- 8/RConn3
  28/RConn3 -- TL<26>-<28>/RConn3 -- TL<28>-<29>/LConn3
  TL<13>-<14>/LConn2 -- 14/LConn2
  TL<15>-<16>/RConn1 -- 15/LConn1
  6/LConn2 -- 5-6 14 km/RConn2 -- TL<6>-<11>/LConn2
  TL<1>-<2>/RConn1 -- 1/LConn1
  TL<6>-<7>/RConn1 -- 7/RConn1
  10-11 14 km/LConn2 -- 11/RConn2
  TL<1>-<39>/LConn2 -- 1/RConn2
  32/LConn2 -- T2: 900MVA 20 kV/230 kV6/LConn2
  load12/LConn2 -- 12/LConn2
  TL<26>--<27>/RConn2 -- load27/LConn2 -- 27/LConn2
  dummy D-Y xfo 20kV/345kV/RConn1 -- 39/RConn1
  TL<2>-<25>/RConn2 -- TL<2>-<3>1/RConn2 -- T2: 900MVA 20 kV/230 kV2/RConn2 -- 2/LConn2
  TL<4>-<5>/RConn3 -- 5/LConn3
  load31/LConn2 -- 31/RConn2 -- G2/RConn2
  T2: 900MVA 20 kV/230 kV4/LConn2 -- TL<3>-<4>2/LConn2 -- TL<6>-<11>/RConn2 -- 11/LConn2
  26/RConn1 -- TL<25>-<26>/RConn1 -- TL<26>--<27>/LConn1
  TL<17>-<18>/RConn3 -- 17/RConn3
  31/LConn1 -- T2: 900MVA 20 kV/230 kV3/LConn1
  37/RConn3 -- T2: 900MVA 20 kV/230 kV1/LConn3
  T2: 900MVA 20 kV/230 kV10/LConn2 -- 21/RConn2
  3/RConn1 -- load3/LConn1 -- TL<3>-<4>/LConn1
  TL<17>-<27>/LConn2 -- 27/RConn2
  25/LConn1 -- TL<25>-<26>/LConn1 -- T2: 900MVA 20 kV/230 kV1/RConn1
  22/RConn2 -- TL<22>-<23>/LConn2 -- T2: 900MVA 20 kV/230 kV11/RConn2
  T2: 900MVA 20 kV/230 kV8/LConn3 -- 19/RConn3
  T2: 900MVA 20 kV/230 kV7/LConn3 -- 38/LConn3
  36/LConn1 -- TL<24>-<23>/RConn1 -- TL<22>-<23>/RConn1
  TL<17>-<27>/LConn3 -- 27/RConn3
  TL<21>-<22>/RConn2 -- 22/LConn2
  TL<17>-<18>/RConn1 -- 17/RConn1
  18/RConn1 -- TL<3>-<18>/RConn1 -- TL<17>-<18>/LConn1
  T2: 900MVA 20 kV/230 kV7/LConn2 -- 38/LConn2
  TL<17>-<18>/RConn2 -- 17/RConn2
  G8/RConn1 -- 37/LConn1
  G8/RConn2 -- 37/LConn2
  G8/RConn3 -- 37/LConn3
  30/LConn1 -- G10/RConn1
  G10/RConn2 -- 30/LConn2
  G10/RConn3 -- 30/LConn3
  38/RConn2 -- G9/RConn2
  38/RConn3 -- G9/RConn3
  38/RConn1 -- G9/RConn1
  G3/RConn2 -- 32/RConn2
  G3/RConn3 -- 32/RConn3
  G3/RConn1 -- 32/RConn1
  G5/RConn2 -- 34/RConn2
  G5/RConn3 -- 34/RConn3
  G5/RConn1 -- 34/RConn1
  G6/RConn2 -- 35./RConn2
  35./RConn3 -- G6/RConn3
  35./RConn1 -- G6/RConn1
  24/RConn1 -- dummy D-Y xfo 20kV/345kV/LConn1
  24/RConn2 -- dummy D-Y xfo 20kV/345kV/LConn2
  24/RConn3 -- dummy D-Y xfo 20kV/345kV/LConn3
  G7/RConn2 -- 35/RConn2
  35/RConn3 -- G7/RConn3
  35/RConn1 -- G7/RConn1
  21/LConn1 -- G4/RConn1
  G4/RConn2 -- 21/LConn2
  21/LConn3 -- G4/RConn3
  G1/RConn3 -- 24/LConn1
  G1/RConn2 -- 24/LConn2
  G1/RConn1 -- 24/LConn3
  41/RConn1 -- T2: 900MVA 20 kV/230 kV7/RConn1
  41/RConn2 -- T2: 900MVA 20 kV/230 kV7/RConn2
  41/RConn3 -- T2: 900MVA 20 kV/230 kV7/RConn3
  41/LConn1 -- TL<26>-<28>1/LConn1
  41/LConn2 -- TL<26>-<28>1/LConn2
  41/LConn3 -- TL<26>-<28>1/LConn3
  29/LConn1 -- TL<26>-<28>2/LConn1
  29/LConn2 -- TL<26>-<28>2/LConn2
  29/LConn3 -- TL<26>-<28>2/LConn3
  40/RConn1 -- TL<26>-<28>2/RConn1
  40/RConn2 -- TL<26>-<28>2/RConn2
  40/RConn3 -- TL<26>-<28>2/RConn3
  Three-Phase Breaker/LConn1 -- TL<26>-<28>1/RConn1
  Three-Phase Breaker/LConn2 -- TL<26>-<28>1/RConn2
  Three-Phase Breaker/RConn1 -- 40/LConn1
  Three-Phase Breaker/RConn2 -- 40/LConn2
  Three-Phase Breaker/RConn3 -- 40/LConn3
  Three-Phase Breaker/LConn3 -- TL<26>-<28>1/RConn3
  TL<2>-<3>1/LConn2 -- 4 WT/LConn2
  TL<2>-<3>1/LConn1 -- 4 WT/LConn1
  TL<2>-<3>1/LConn3 -- 4 WT/LConn3
  TL<3>-<4>1/LConn1 -- 4 WT/LConn4
  TL<3>-<4>1/LConn2 -- 4 WT/LConn5
  TL<3>-<4>1/LConn3 -- 4 WT/LConn6
  TL<3>-<4>2/RConn1 -- 4 WT/RConn1
  TL<3>-<4>2/RConn2 -- 4 WT/RConn2
  TL<3>-<4>2/RConn3 -- 4 WT/RConn3
  4 WT/RConn4 -- TL<3>-<4>3/RConn1
  4 WT/RConn5 -- TL<3>-<4>3/RConn2
  4 WT/RConn6 -- TL<3>-<4>3/RConn3
